simulink library "DAMA_lib"  (Simulink 6.6)
undefined symbols (not defined in the file or in its folder): aa2rot, D, DiscIntNeverNeededParam, DRprogressbar, epsilon, Kd, Ko, Kp, manip, manipulator, path_des, Q, q0, q_d0, rho, robot, show_3D, StartTime, subs, Ts, VR_handle, vrmfunc
libraries: DAMA_lib x7, vrlib x1, simulink x1
(part 3 of 4)

== system DAMA_lib/Kinematics/Transpose Jacobian Inverse Kinematics/Subsystem/Subsystem1 ==
  nsa_e_d_V : Inport
  Mux : Mux  Inputs=3
  invL1 : Fcn  Expr=2*(u(10)^2*u(1)^2+u(13)^2*u(4)^2+u(16)^2*u(7)^2+u(12)*u(3)*u(10)*u(1)+u(12)*u(3)*u(14)*u(5)+u(12)*u(3)*u(13)*u(4)+u(12)*u(3)*u(17)*u(8)+u(12)*u(3)*u(16)*u(7)+u(10)*u(1)*u(11)*u(2)+u(10)*u(1)*u(14)*u(5)+2*u(10)*u(1)*u(13)*u(4)+u(10)*u(1)*u(17)*u(8)+2*u(10)*u(1)*u(16)*u(7)+u(15)*u(6)*u(11)*u(2)+u(15)*u(6)*u(10)*u(1)+u(15)*u(6)*u(13)*u(4)+u(15)*u(6)*u(17)*u(8)+u(15)*u(6)*u(16)*u(7)+u(13)*u(4)*u(11)*u(2)+u(13)*u(4)*u(14)*u(5)+u(13)*u(4)*u(17)*u(8)+2*u(13)*u(4)*u(16)*u(7)+u(18)*u(9)*u(11)*u(2)+u(18)*u(9)*u(10)*u(1)+u(18)*u(9)*u(14)*u(5)+u(18)*u(9)*u(13)*u(4)+u(18)*u(9)*u(16)*u(7)+u(16)*u(7)*u(11)*u(2)+u(16)*u(7)*u(14)*u(5)+u(16)*u(7)*u(17)*u(8)-u(12)*u(2)*u(14)*u(6)-u(12)*u(2)*u(17)*u(9)-u(15)*u(5)*u(11)*u(3)-u(15)*u(5)*u(17)*u(9)-u(18)*u(8)*u(11)*u(3)-u(18)*u(8)*u(14)*u(6))/(u(12)*u(3)*u(13)^2*u(4)^2+u(12)*u(3)*u(16)^2*u(7)^2+u(12)^2*u(3)^2*u(14)*u(5)+u(12)^2*u(3)^2*u(13)*u(4)+u(12)^2*u(3)^2*u(17)*u(8)+u(12)^2*u(3)^2*u(16)*u(7)+u(11)*u(2)*u(13)^2*u(4)^2+u(11)*u(2)*u(16)^2*u(7)^2+u(11)^2*u(2)^2*u(15)*u(6)+u(11)^2*u(2)^2*u(13)*u(4)+u(11)^2*u(2)^2*u(18)*u(9)+u(11)^2*u(2)^2*u(16)*u(7)+u(15)*u(6)*u(10)^2*u(1)^2+u(15)*u(6)*u(16)^2*u(7)^2+u(15)^2*u(6)^2*u(11)*u(2)+u(15)^2*u(6)^2*u(10)*u(1)+u(15)^2*u(6)^2*u(17)*u(8)+u(15)^2*u(6)^2*u(16)*u(7)+u(14)*u(5)*u(10)^2*u(1)^2+u(14)*u(5)*u(16)^2*u(7)^2+u(14)^2*u(5)^2*u(12)*u(3)+u(14)^2*u(5)^2*u(10)*u(1)+u(14)^2*u(5)^2*u(18)*u(9)+u(14)^2*u(5)^2*u(16)*u(7)+u(18)*u(9)*u(10)^2*u(1)^2+u(18)*u(9)*u(13)^2*u(4)^2+u(18)^2*u(9)^2*u(11)*u(2)+u(18)^2*u(9)^2*u(10)*u(1)+u(18)^2*u(9)^2*u(14)*u(5)+u(18)^2*u(9)^2*u(13)*u(4)+u(17)*u(8)*u(10)^2*u(1)^2+u(17)*u(8)*u(13)^2*u(4)^2+u(17)^2*u(8)^2*u(12)*u(3)+u(17)^2*u(8)^2*u(10)*u(1)+u(17)^2*u(8)^2*u(15)*u(6)+u(17)^2*u(8)^2*u(13)*u(4)-u(10)*u(2)*u(14)^2*u(4)*u(5)-u(10)*u(2)*u(14)*u(4)^2*u(13)-u(10)*u(2)*u(17)*u(7)^2*u(16)-u(10)*u(2)*u(17)^2*u(7)*u(8)-u(10)*u(2)^2*u(14)*u(4)*u(11)+2*u(12)*u(3)*u(10)*u(1)*u(14)*u(5)+u(12)*u(3)*u(10)*u(1)*u(13)*u(4)+2*u(12)*u(3)*u(10)*u(1)*u(17)*u(8)+u(12)*u(3)*u(10)*u(1)*u(16)*u(7)+u(12)*u(3)*u(15)*u(6)*u(11)*u(2)+u(12)*u(3)*u(15)*u(6)*u(10)*u(1)+u(12)*u(3)*u(15)*u(6)*u(13)*u(4)+2*u(12)*u(3)*u(15)*u(6)*u(17)*u(8)+2*u(12)*u(3)*u(15)*u(6)*u(16)*u(7)+2*u(12)*u(3)*u(13)*u(4)*u(11)*u(2)+2*u(12)*u(3)*u(13)*u(4)*u(14)*u(5)+2*u(12)*u(3)*u(13)*u(4)*u(17)*u(8)+2*u(12)*u(3)*u(13)*u(4)*u(16)*u(7)+u(12)*u(3)*u(18)*u(9)*u(11)*u(2)+u(12)*u(3)*u(18)*u(9)*u(10)*u(1)+2*u(12)*u(3)*u(18)*u(9)*u(14)*u(5)+2*u(12)*u(3)*u(18)*u(9)*u(13)*u(4)+u(12)*u(3)*u(18)*u(9)*u(16)*u(7)+2*u(12)*u(3)*u(16)*u(7)*u(11)*u(2)+2*u(12)*u(3)*u(16)*u(7)*u(14)*u(5)+2*u(12)*u(3)*u(16)*u(7)*u(17)*u(8)-u(12)^2*u(3)*u(2)*u(14)*u(6)-u(12)^2*u(3)*u(2)*u(17)*u(9)-u(12)*u(3)^2*u(15)*u(5)*u(11)-u(12)*u(3)*u(15)*u(5)*u(17)*u(9)-u(12)*u(3)^2*u(18)*u(8)*u(11)-u(12)*u(3)*u(18)*u(8)*u(14)*u(6)+u(11)*u(2)*u(12)*u(3)*u(14)*u(5)+u(11)*u(2)*u(12)*u(3)*u(17)*u(8)+u(11)*u(2)*u(10)*u(1)*u(14)*u(5)+u(11)*u(2)*u(10)*u(1)*u(13)*u(4)+u(11)*u(2)*u(10)*u(1)*u(17)*u(8)+u(11)*u(2)*u(10)*u(1)*u(16)*u(7)+2*u(11)*u(2)*u(15)*u(6)*u(10)*u(1)+2*u(11)*u(2)*u(15)*u(6)*u(13)*u(4)+2*u(11)*u(2)*u(15)*u(6)*u(17)*u(8)+2*u(11)*u(2)*u(15)*u(6)*u(16)*u(7)+u(11)*u(2)*u(13)*u(4)*u(14)*u(5)+2*u(11)*u(2)*u(13)*u(4)*u(17)*u(8)+2*u(11)*u(2)*u(13)*u(4)*u(16)*u(7)+2*u(11)*u(2)*u(18)*u(9)*u(10)*u(1)+2*u(11)*u(2)*u(18)*u(9)*u(14)*u(5)+2*u(11)*u(2)*u(18)*u(9)*u(13)*u(4)+2*u(11)*u(2)*u(18)*u(9)*u(16)*u(7)+2*u(11)*u(2)*u(16)*u(7)*u(14)*u(5)+u(11)*u(2)*u(16)*u(7)*u(17)*u(8)-u(11)*u(2)^2*u(12)*u(14)*u(6)-u(11)*u(2)^2*u(12)*u(17)*u(9)-u(11)^2*u(2)*u(15)*u(5)*u(3)-u(11)*u(2)*u(15)*u(5)*u(17)*u(9)-u(11)^2*u(2)*u(18)*u(8)*u(3)-u(11)*u(2)*u(18)*u(8)*u(14)*u(6)+u(15)*u(6)*u(12)*u(3)*u(14)*u(5)+2*u(15)*u(6)*u(10)*u(1)*u(14)*u(5)+u(15)*u(6)*u(10)*u(1)*u(13)*u(4)+2*u(15)*u(6)*u(10)*u(1)*u(17)*u(8)+2*u(15)*u(6)*u(10)*u(1)*u(16)*u(7)+2*u(15)*u(6)*u(13)*u(4)*u(17)*u(8)+u(15)*u(6)*u(13)*u(4)*u(16)*u(7)+2*u(15)*u(6)*u(18)*u(9)*u(11)*u(2)+2*u(15)*u(6)*u(18)*u(9)*u(10)*u(1)+u(15)*u(6)*u(18)*u(9)*u(14)*u(5)+u(15)*u(6)*u(18)*u(9)*u(13)*u(4)+u(15)*u(6)*u(18)*u(9)*u(16)*u(7)+2*u(15)*u(6)*u(16)*u(7)*u(14)*u(5)+2*u(15)*u(6)*u(16)*u(7)*u(17)*u(8)-u(15)*u(6)^2*u(12)*u(2)*u(14)-u(15)*u(6)*u(12)*u(2)*u(17)*u(9)-u(15)^2*u(6)*u(5)*u(11)*u(3)-u(15)^2*u(6)*u(5)*u(17)*u(9)-u(15)*u(6)*u(18)*u(8)*u(11)*u(3)-u(15)*u(6)^2*u(18)*u(8)*u(14)+2*u(14)*u(5)*u(12)*u(3)*u(17)*u(8)+u(14)*u(5)*u(10)*u(1)*u(13)*u(4)+2*u(14)*u(5)*u(10)*u(1)*u(17)*u(8)+2*u(14)*u(5)*u(10)*u(1)*u(16)*u(7)+u(14)*u(5)*u(15)*u(6)*u(11)*u(2)+u(14)*u(5)*u(15)*u(6)*u(17)*u(8)+u(14)*u(5)*u(13)*u(4)*u(17)*u(8)+u(14)*u(5)*u(13)*u(4)*u(16)*u(7)+2*u(14)*u(5)*u(18)*u(9)*u(10)*u(1)+2*u(14)*u(5)*u(18)*u(9)*u(13)*u(4)+2*u(14)*u(5)*u(18)*u(9)*u(16)*u(7)+u(14)*u(5)*u(16)*u(7)*u(17)*u(8)-u(14)^2*u(5)*u(12)*u(2)*u(6)-u(14)*u(5)*u(12)*u(2)*u(17)*u(9)-u(14)*u(5)^2*u(15)*u(11)*u(3)-u(14)*u(5)^2*u(15)*u(17)*u(9)-u(14)*u(5)*u(18)*u(8)*u(11)*u(3)-u(14)^2*u(5)*u(18)*u(8)*u(6)+u(18)*u(9)*u(12)*u(3)*u(17)*u(8)+2*u(18)*u(9)*u(10)*u(1)*u(13)*u(4)+2*u(18)*u(9)*u(10)*u(1)*u(17)*u(8)+u(18)*u(9)*u(10)*u(1)*u(16)*u(7)+u(18)*u(9)*u(15)*u(6)*u(17)*u(8)+2*u(18)*u(9)*u(13)*u(4)*u(17)*u(8)+u(18)*u(9)*u(13)*u(4)*u(16)*u(7)-u(18)*u(9)*u(12)*u(2)*u(14)*u(6)-u(18)*u(9)^2*u(12)*u(2)*u(17)-u(18)*u(9)*u(15)*u(5)*u(11)*u(3)-u(18)*u(9)^2*u(15)*u(5)*u(17)-u(18)^2*u(9)*u(8)*u(11)*u(3)-u(18)^2*u(9)*u(8)*u(14)*u(6)+2*u(17)*u(8)*u(10)*u(1)*u(13)*u(4)+u(17)*u(8)*u(10)*u(1)*u(16)*u(7)+u(17)*u(8)*u(13)*u(4)*u(16)*u(7)+u(17)*u(8)*u(18)*u(9)*u(11)*u(2)+u(17)*u(8)*u(18)*u(9)*u(14)*u(5)-u(17)*u(8)*u(12)*u(2)*u(14)*u(6)-u(17)^2*u(8)*u(12)*u(2)*u(9)-u(17)*u(8)*u(15)*u(5)*u(11)*u(3)-u(17)^2*u(8)*u(15)*u(5)*u(9)-u(17)*u(8)^2*u(18)*u(11)*u(3)-u(17)*u(8)^2*u(18)*u(14)*u(6)-u(10)^2*u(2)*u(14)*u(4)*u(1)-u(10)*u(2)*u(14)*u(4)*u(17)*u(8)-u(10)*u(2)*u(14)*u(4)*u(16)*u(7)-u(10)*u(2)^2*u(17)*u(7)*u(11)-u(10)^2*u(2)*u(17)*u(7)*u(1)-u(10)*u(2)*u(17)*u(7)*u(14)*u(5)-u(10)*u(2)*u(17)*u(7)*u(13)*u(4)-u(10)*u(2)*u(12)*u(1)*u(14)*u(6)-u(10)*u(2)*u(12)*u(1)*u(17)*u(9)-u(10)*u(2)*u(15)*u(4)*u(11)*u(3)-u(10)*u(2)*u(15)*u(4)*u(14)*u(6)-u(10)*u(2)*u(15)*u(4)*u(17)*u(9)-u(10)*u(2)*u(18)*u(7)*u(11)*u(3)-u(10)*u(2)*u(18)*u(7)*u(14)*u(6)-u(10)*u(2)*u(18)*u(7)*u(17)*u(9)-u(13)*u(5)*u(11)^2*u(1)*u(2)-u(13)*u(5)*u(11)*u(1)^2*u(10)-u(13)*u(5)*u(17)*u(7)^2*u(16)-u(13)*u(5)*u(17)^2*u(7)*u(8)-u(13)*u(5)^2*u(11)*u(1)*u(14)-u(13)^2*u(5)*u(11)*u(1)*u(4)-u(13)*u(5)*u(11)*u(1)*u(17)*u(8)-u(13)*u(5)*u(11)*u(1)*u(16)*u(7)-u(13)*u(5)*u(17)*u(7)*u(11)*u(2)-u(13)*u(5)*u(17)*u(7)*u(10)*u(1)-u(13)*u(5)^2*u(17)*u(7)*u(14)-u(13)^2*u(5)*u(17)*u(7)*u(4)-u(13)*u(5)*u(12)*u(1)*u(11)*u(3)-u(13)*u(5)*u(12)*u(1)*u(14)*u(6)-u(13)*u(5)*u(12)*u(1)*u(17)*u(9)-u(13)*u(5)*u(15)*u(4)*u(11)*u(3)-u(13)*u(5)*u(15)*u(4)*u(17)*u(9)-u(13)*u(5)*u(18)*u(7)*u(11)*u(3)-u(13)*u(5)*u(18)*u(7)*u(14)*u(6)-u(13)*u(5)*u(18)*u(7)*u(17)*u(9)-u(16)*u(8)*u(14)^2*u(4)*u(5)-u(16)*u(8)*u(11)^2*u(1)*u(2)-u(16)*u(8)*u(14)*u(4)^2*u(13)-u(16)*u(8)*u(11)*u(1)^2*u(10)-u(16)*u(8)*u(11)*u(1)*u(14)*u(5)-u(16)*u(8)*u(11)*u(1)*u(13)*u(4)-u(16)*u(8)^2*u(11)*u(1)*u(17)-u(16)^2*u(8)*u(11)*u(1)*u(7)-u(16)*u(8)*u(14)*u(4)*u(11)*u(2)-u(16)*u(8)*u(14)*u(4)*u(10)*u(1)-u(16)*u(8)^2*u(14)*u(4)*u(17)-u(16)^2*u(8)*u(14)*u(4)*u(7)-u(16)*u(8)*u(12)*u(1)*u(11)*u(3)-u(16)*u(8)*u(12)*u(1)*u(14)*u(6)-u(16)*u(8)*u(12)*u(1)*u(17)*u(9)-u(16)*u(8)*u(15)*u(4)*u(11)*u(3)-u(16)*u(8)*u(15)*u(4)*u(14)*u(6)-u(16)*u(8)*u(15)*u(4)*u(17)*u(9)-u(16)*u(8)*u(18)*u(7)*u(11)*u(3)-u(16)*u(8)*u(18)*u(7)*u(14)*u(6)-u(10)*u(3)*u(15)^2*u(4)*u(6)-u(10)*u(3)*u(15)*u(4)^2*u(13)-u(10)*u(3)*u(18)^2*u(7)*u(9)-u(10)*u(3)*u(18)*u(7)^2*u(16)-u(10)*u(3)*u(11)*u(1)*u(15)*u(5)-u(10)*u(3)*u(11)*u(1)*u(18)*u(8)-u(10)*u(3)*u(14)*u(4)*u(12)*u(2)-u(10)*u(3)*u(14)*u(4)*u(15)*u(5)-u(10)*u(3)*u(14)*u(4)*u(18)*u(8)-u(10)*u(3)*u(17)*u(7)*u(12)*u(2)-u(10)*u(3)*u(17)*u(7)*u(15)*u(5)-u(10)*u(3)*u(17)*u(7)*u(18)*u(8)-u(10)*u(3)^2*u(15)*u(4)*u(12)-u(10)^2*u(3)*u(15)*u(4)*u(1)-u(10)*u(3)*u(15)*u(4)*u(18)*u(9)-u(10)*u(3)*u(15)*u(4)*u(16)*u(7)-u(10)*u(3)^2*u(18)*u(7)*u(12)-u(10)^2*u(3)*u(18)*u(7)*u(1)-u(10)*u(3)*u(18)*u(7)*u(15)*u(6)-u(10)*u(3)*u(18)*u(7)*u(13)*u(4)-u(13)*u(6)*u(12)*u(1)^2*u(10)-u(13)*u(6)*u(12)^2*u(1)*u(3)-u(13)*u(6)*u(18)^2*u(7)*u(9)-u(13)*u(6)*u(18)*u(7)^2*u(16)-u(13)*u(6)*u(11)*u(1)*u(12)*u(2)-u(13)*u(6)*u(11)*u(1)*u(15)*u(5)-u(13)*u(6)*u(11)*u(1)*u(18)*u(8)-u(13)*u(6)*u(14)*u(4)*u(12)*u(2)-u(13)*u(6)*u(14)*u(4)*u(18)*u(8)-u(13)*u(6)*u(17)*u(7)*u(12)*u(2)-u(13)*u(6)*u(17)*u(7)*u(15)*u(5)-u(13)*u(6)*u(17)*u(7)*u(18)*u(8)-u(13)*u(6)^2*u(12)*u(1)*u(15)-u(13)^2*u(6)*u(12)*u(1)*u(4)-u(13)*u(6)*u(12)*u(1)*u(18)*u(9)-u(13)*u(6)*u(12)*u(1)*u(16)*u(7)-u(13)*u(6)*u(18)*u(7)*u(12)*u(3)-u(13)*u(6)*u(18)*u(7)*u(10)*u(1)-u(13)*u(6)^2*u(18)*u(7)*u(15)-u(13)^2*u(6)*u(18)*u(7)*u(4)-u(16)*u(9)*u(12)*u(1)^2*u(10)-u(16)*u(9)*u(12)^2*u(1)*u(3)-u(16)*u(9)*u(15)^2*u(4)*u(6)-u(16)*u(9)*u(15)*u(4)^2*u(13)-u(16)*u(9)*u(11)*u(1)*u(12)*u(2)-u(16)*u(9)*u(11)*u(1)*u(15)*u(5)-u(16)*u(9)*u(11)*u(1)*u(18)*u(8)-u(16)*u(9)*u(14)*u(4)*u(12)*u(2)-u(16)*u(9)*u(14)*u(4)*u(15)*u(5)-u(16)*u(9)*u(14)*u(4)*u(18)*u(8)-u(16)*u(9)*u(17)*u(7)*u(12)*u(2)-u(16)*u(9)*u(17)*u(7)*u(15)*u(5)-u(16)*u(9)*u(12)*u(1)*u(15)*u(6)-u(16)*u(9)*u(12)*u(1)*u(13)*u(4)-u(16)*u(9)^2*u(12)*u(1)*u(18)-u(16)^2*u(9)*u(12)*u(1)*u(7)-u(16)*u(9)*u(15)*u(4)*u(12)*u(3)-u(16)*u(9)*u(15)*u(4)*u(10)*u(1)-u(16)*u(9)^2*u(15)*u(4)*u(18)-u(16)^2*u(9)*u(15)*u(4)*u(7))*u(19)+2*(u(14)^2*u(4)*u(5)+u(11)^2*u(1)*u(2)+u(14)*u(4)^2*u(13)+u(11)*u(1)^2*u(10)+u(17)*u(7)^2*u(16)+u(17)^2*u(7)*u(8)+u(11)*u(1)*u(14)*u(5)+u(11)*u(1)*u(13)*u(4)+u(11)*u(1)*u(17)*u(8)+u(11)*u(1)*u(16)*u(7)+u(14)*u(4)*u(11)*u(2)+u(14)*u(4)*u(10)*u(1)+u(14)*u(4)*u(17)*u(8)+u(14)*u(4)*u(16)*u(7)+u(17)*u(7)*u(11)*u(2)+u(17)*u(7)*u(10)*u(1)+u(17)*u(7)*u(14)*u(5)+u(17)*u(7)*u(13)*u(4)+u(12)*u(1)*u(11)*u(3)+u(12)*u(1)*u(14)*u(6)+u(12)*u(1)*u(17)*u(9)+u(15)*u(4)*u(11)*u(3)+u(15)*u(4)*u(14)*u(6)+u(15)*u(4)*u(17)*u(9)+u(18)*u(7)*u(11)*u(3)+u(18)*u(7)*u(14)*u(6)+u(18)*u(7)*u(17)*u(9))/(u(12)*u(3)*u(13)^2*u(4)^2+u(12)*u(3)*u(16)^2*u(7)^2+u(12)^2*u(3)^2*u(14)*u(5)+u(12)^2*u(3)^2*u(13)*u(4)+u(12)^2*u(3)^2*u(17)*u(8)+u(12)^2*u(3)^2*u(16)*u(7)+u(11)*u(2)*u(13)^2*u(4)^2+u(11)*u(2)*u(16)^2*u(7)^2+u(11)^2*u(2)^2*u(15)*u(6)+u(11)^2*u(2)^2*u(13)*u(4)+u(11)^2*u(2)^2*u(18)*u(9)+u(11)^2*u(2)^2*u(16)*u(7)+u(15)*u(6)*u(10)^2*u(1)^2+u(15)*u(6)*u(16)^2*u(7)^2+u(15)^2*u(6)^2*u(11)*u(2)+u(15)^2*u(6)^2*u(10)*u(1)+u(15)^2*u(6)^2*u(17)*u(8)+u(15)^2*u(6)^2*u(16)*u(7)+u(14)*u(5)*u(10)^2*u(1)^2+u(14)*u(5)*u(16)^2*u(7)^2+u(14)^2*u(5)^2*u(12)*u(3)+u(14)^2*u(5)^2*u(10)*u(1)+u(14)^2*u(5)^2*u(18)*u(9)+u(14)^2*u(5)^2*u(16)*u(7)+u(18)*u(9)*u(10)^2*u(1)^2+u(18)*u(9)*u(13)^2*u(4)^2+u(18)^2*u(9)^2*u(11)*u(2)+u(18)^2*u(9)^2*u(10)*u(1)+u(18)^2*u(9)^2*u(14)*u(5)+u(18)^2*u(9)^2*u(13)*u(4)+u(17)*u(8)*u(10)^2*u(1)^2+u(17)*u(8)*u(13)^2*u(4)^2+u(17)^2*u(8)^2*u(12)*u(3)+u(17)^2*u(8)^2*u(10)*u(1)+u(17)^2*u(8)^2*u(15)*u(6)+u(17)^2*u(8)^2*u(13)*u(4)-u(10)*u(2)*u(14)^2*u(4)*u(5)-u(10)*u(2)*u(14)*u(4)^2*u(13)-u(10)*u(2)*u(17)*u(7)^2*u(16)-u(10)*u(2)*u(17)^2*u(7)*u(8)-u(10)*u(2)^2*u(14)*u(4)*u(11)+2*u(12)*u(3)*u(10)*u(1)*u(14)*u(5)+u(12)*u(3)*u(10)*u(1)*u(13)*u(4)+2*u(12)*u(3)*u(10)*u(1)*u(17)*u(8)+u(12)*u(3)*u(10)*u(1)*u(16)*u(7)+u(12)*u(3)*u(15)*u(6)*u(11)*u(2)+u(12)*u(3)*u(15)*u(6)*u(10)*u(1)+u(12)*u(3)*u(15)*u(6)*u(13)*u(4)+2*u(12)*u(3)*u(15)*u(6)*u(17)*u(8)+2*u(12)*u(3)*u(15)*u(6)*u(16)*u(7)+2*u(12)*u(3)*u(13)*u(4)*u(11)*u(2)+2*u(12)*u(3)*u(13)*u(4)*u(14)*u(5)+2*u(12)*u(3)*u(13)*u(4)*u(17)*u(8)+2*u(12)*u(3)*u(13)*u(4)*u(16)*u(7)+u(12)*u(3)*u(18)*u(9)*u(11)*u(2)+u(12)*u(3)*u(18)*u(9)*u(10)*u(1)+2*u(12)*u(3)*u(18)*u(9)*u(14)*u(5)+2*u(12)*u(3)*u(18)*u(9)*u(13)*u(4)+u(12)*u(3)*u(18)*u(9)*u(16)*u(7)+2*u(12)*u(3)*u(16)*u(7)*u(11)*u(2)+2*u(12)*u(3)*u(16)*u(7)*u(14)*u(5)+2*u(12)*u(3)*u(16)*u(7)*u(17)*u(8)-u(12)^2*u(3)*u(2)*u(14)*u(6)-u(12)^2*u(3)*u(2)*u(17)*u(9)-u(12)*u(3)^2*u(15)*u(5)*u(11)-u(12)*u(3)*u(15)*u(5)*u(17)*u(9)-u(12)*u(3)^2*u(18)*u(8)*u(11)-u(12)*u(3)*u(18)*u(8)*u(14)*u(6)+u(11)*u(2)*u(12)*u(3)*u(14)*u(5)+u(11)*u(2)*u(12)*u(3)*u(17)*u(8)+u(11)*u(2)*u(10)*u(1)*u(14)*u(5)+u(11)*u(2)*u(10)*u(1)*u(13)*u(4)+u(11)*u(2)*u(10)*u(1)*u(17)*u(8)+u(11)*u(2)*u(10)*u(1)*u(16)*u(7)+2*u(11)*u(2)*u(15)*u(6)*u(10)*u(1)+2*u(11)*u(2)*u(15)*u(6)*u(13)*u(4)+2*u(11)*u(2)*u(15)*u(6)*u(17)*u(8)+2*u(11)*u(2)*u(15)*u(6)*u(16)*u(7)+u(11)*u(2)*u(13)*u(4)*u(14)*u(5)+2*u(11)*u(2)*u(13)*u(4)*u(17)*u(8)+2*u(11)*u(2)*u(13)*u(4)*u(16)*u(7)+2*u(11)*u(2)*u(18)*u(9)*u(10)*u(1)+2*u(11)*u(2)*u(18)*u(9)*u(14)*u(5)+2*u(11)*u(2)*u(18)*u(9)*u(13)*u(4)+2*u(11)*u(2)*u(18)*u(9)*u(16)*u(7)+2*u(11)*u(2)*u(16)*u(7)*u(14)*u(5)+u(11)*u(2)*u(16)*u(7)*u(17)*u(8)-u(11)*u(2)^2*u(12)*u(14)*u(6)-u(11)*u(2)^2*u(12)*u(17)*u(9)-u(11)^2*u(2)*u(15)*u(5)*u(3)-u(11)*u(2)*u(15)*u(5)*u(17)*u(9)-u(11)^2*u(2)*u(18)*u(8)*u(3)-u(11)*u(2)*u(18)*u(8)*u(14)*u(6)+u(15)*u(6)*u(12)*u(3)*u(14)*u(5)+2*u(15)*u(6)*u(10)*u(1)*u(14)*u(5)+u(15)*u(6)*u(10)*u(1)*u(13)*u(4)+2*u(15)*u(6)*u(10)*u(1)*u(17)*u(8)+2*u(15)*u(6)*u(10)*u(1)*u(16)*u(7)+2*u(15)*u(6)*u(13)*u(4)*u(17)*u(8)+u(15)*u(6)*u(13)*u(4)*u(16)*u(7)+2*u(15)*u(6)*u(18)*u(9)*u(11)*u(2)+2*u(15)*u(6)*u(18)*u(9)*u(10)*u(1)+u(15)*u(6)*u(18)*u(9)*u(14)*u(5)+u(15)*u(6)*u(18)*u(9)*u(13)*u(4)+u(15)*u(6)*u(18)*u(9)*u(16)*u(7)+2*u(15)*u(6)*u(16)*u(7)*u(14)*u(5)+2*u(15)*u(6)*u(16)*u(7)*u(17)*u(8)-u(15)*u(6)^2*u(12)*u(2)*u(14)-u(15)*u(6)*u(12)*u(2)*u(17)*u(9)-u(15)^2*u(6)*u(5)*u(11)*u(3)-u(15)^2*u(6)*u(5)*u(17)*u(9)-u(15)*u(6)*u(18)*u(8)*u(11)*u(3)-u(15)*u(6)^2*u(18)*u(8)*u(14)+2*u(14)*u(5)*u(12)*u(3)*u(17)*u(8)+u(14)*u(5)*u(10)*u(1)*u(13)*u(4)+2*u(14)*u(5)*u(10)*u(1)*u(17)*u(8)+2*u(14)*u(5)*u(10)*u(1)*u(16)*u(7)+u(14)*u(5)*u(15)*u(6)*u(11)*u(2)+u(14)*u(5)*u(15)*u(6)*u(17)*u(8)+u(14)*u(5)*u(13)*u(4)*u(17)*u(8)+u(14)*u(5)*u(13)*u(4)*u(16)*u(7)+2*u(14)*u(5)*u(18)*u(9)*u(10)*u(1)+2*u(14)*u(5)*u(18)*u(9)*u(13)*u(4)+2*u(14)*u(5)*u(18)*u(9)*u(16)*u(7)+u(14)*u(5)*u(16)*u(7)*u(17)*u(8)-u(14)^2*u(5)*u(12)*u(2)*u(6)-u(14)*u(5)*u(12)*u(2)*u(17)*u(9)-u(14)*u(5)^2*u(15)*u(11)*u(3)-u(14)*u(5)^2*u(15)*u(17)*u(9)-u(14)*u(5)*u(18)*u(8)*u(11)*u(3)-u(14)^2*u(5)*u(18)*u(8)*u(6)+u(18)*u(9)*u(12)*u(3)*u(17)*u(8)+2*u(18)*u(9)*u(10)*u(1)*u(13)*u(4)+2*u(18)*u(9)*u(10)*u(1)*u(17)*u(8)+u(18)*u(9)*u(10)*u(1)*u(16)*u(7)+u(18)*u(9)*u(15)*u(6)*u(17)*u(8)+2*u(18)*u(9)*u(13)*u(4)*u(17)*u(8)+u(18)*u(9)*u(13)*u(4)*u(16)*u(7)-u(18)*u(9)*u(12)*u(2)*u(14)*u(6)-u(18)*u(9)^2*u(12)*u(2)*u(17)-u(18)*u(9)*u(15)*u(5)*u(11)*u(3)-u(18)*u(9)^2*u(15)*u(5)*u(17)-u(18)^2*u(9)*u(8)*u(11)*u(3)-u(18)^2*u(9)*u(8)*u(14)*u(6)+2*u(17)*u(8)*u(10)*u(1)*u(13)*u(4)+u(17)*u(8)*u(10)*u(1)*u(16)*u(7)+u(17)*u(8)*u(13)*u(4)*u(16)*u(7)+u(17)*u(8)*u(18)*u(9)*u(11)*u(2)+u(17)*u(8)*u(18)*u(9)*u(14)*u(5)-u(17)*u(8)*u(12)*u(2)*u(14)*u(6)-u(17)^2*u(8)*u(12)*u(2)*u(9)-u(17)*u(8)*u(15)*u(5)*u(11)*u(3)-u(17)^2*u(8)*u(15)*u(5)*u(9)-u(17)*u(8)^2*u(18)*u(11)*u(3)-u(17)*u(8)^2*u(18)*u(14)*u(6)-u(10)^2*u(2)*u(14)*u(4)*u(1)-u(10)*u(2)*u(14)*u(4)*u(17)*u(8)-u(10)*u(2)*u(14)*u(4)*u(16)*u(7)-u(10)*u(2)^2*u(17)*u(7)*u(11)-u(10)^2*u(2)*u(17)*u(7)*u(1)-u(10)*u(2)*u(17)*u(7)*u(14)*u(5)-u(10)*u(2)*u(17)*u(7)*u(13)*u(4)-u(10)*u(2)*u(12)*u(1)*u(14)*u(6)-u(10)*u(2)*u(12)*u(1)*u(17)*u(9)-u(10)*u(2)*u(15)*u(4)*u(11)*u(3)-u(10)*u(2)*u(15)*u(4)*u(14)*u(6)-u(10)*u(2)*u(15)*u(4)*u(17)*u(9)-u(10)*u(2)*u(18)*u(7)*u(11)*u(3)-u(10)*u(2)*u(18)*u(7)*u(14)*u(6)-u(10)*u(2)*u(18)*u(7)*u(17)*u(9)-u(13)*u(5)*u(11)^2*u(1)*u(2)-u(13)*u(5)*u(11)*u(1)^2*u(10)-u(13)*u(5)*u(17)*u(7)^2*u(16)-u(13)*u(5)*u(17)^2*u(7)*u(8)-u(13)*u(5)^2*u(11)*u(1)*u(14)-u(13)^2*u(5)*u(11)*u(1)*u(4)-u(13)*u(5)*u(11)*u(1)*u(17)*u(8)-u(13)*u(5)*u(11)*u(1)*u(16)*u(7)-u(13)*u(5)*u(17)*u(7)*u(11)*u(2)-u(13)*u(5)*u(17)*u(7)*u(10)*u(1)-u(13)*u(5)^2*u(17)*u(7)*u(14)-u(13)^2*u(5)*u(17)*u(7)*u(4)-u(13)*u(5)*u(12)*u(1)*u(11)*u(3)-u(13)*u(5)*u(12)*u(1)*u(14)*u(6)-u(13)*u(5)*u(12)*u(1)*u(17)*u(9)-u(13)*u(5)*u(15)*u(4)*u(11)*u(3)-u(13)*u(5)*u(15)*u(4)*u(17)*u(9)-u(13)*u(5)*u(18)*u(7)*u(11)*u(3)-u(13)*u(5)*u(18)*u(7)*u(14)*u(6)-u(13)*u(5)*u(18)*u(7)*u(17)*u(9)-u(16)*u(8)*u(14)^2*u(4)*u(5)-u(16)*u(8)*u(11)^2*u(1)*u(2)-u(16)*u(8)*u(14)*u(4)^2*u(13)-u(16)*u(8)*u(11)*u(1)^2*u(10)-u(16)*u(8)*u(11)*u(1)*u(14)*u(5)-u(16)*u(8)*u(11)*u(1)*u(13)*u(4)-u(16)*u(8)^2*u(11)*u(1)*u(17)-u(16)^2*u(8)*u(11)*u(1)*u(7)-u(16)*u(8)*u(14)*u(4)*u(11)*u(2)-u(16)*u(8)*u(14)*u(4)*u(10)*u(1)-u(16)*u(8)^2*u(14)*u(4)*u(17)-u(16)^2*u(8)*u(14)*u(4)*u(7)-u(16)*u(8)*u(12)*u(1)*u(11)*u(3)-u(16)*u(8)*u(12)*u(1)*u(14)*u(6)-u(16)*u(8)*u(12)*u(1)*u(17)*u(9)-u(16)*u(8)*u(15)*u(4)*u(11)*u(3)-u(16)*u(8)*u(15)*u(4)*u(14)*u(6)-u(16)*u(8)*u(15)*u(4)*u(17)*u(9)-u(16)*u(8)*u(18)*u(7)*u(11)*u(3)-u(16)*u(8)*u(18)*u(7)*u(14)*u(6)-u(10)*u(3)*u(15)^2*u(4)*u(6)-u(10)*u(3)*u(15)*u(4)^2*u(13)-u(10)*u(3)*u(18)^2*u(7)*u(9)-u(10)*u(3)*u(18)*u(7)^2*u(16)-u(10)*u(3)*u(11)*u(1)*u(15)*u(5)-u(10)*u(3)*u(11)*u(1)*u(18)*u(8)-u(10)*u(3)*u(14)*u(4)*u(12)*u(2)-u(10)*u(3)*u(14)*u(4)*u(15)*u(5)-u(10)*u(3)*u(14)*u(4)*u(18)*u(8)-u(10)*u(3)*u(17)*u(7)*u(12)*u(2)-u(10)*u(3)*u(17)*u(7)*u(15)*u(5)-u(10)*u(3)*u(17)*u(7)*u(18)*u(8)-u(10)*u(3)^2*u(15)*u(4)*u(12)-u(10)^2*u(3)*u(15)*u(4)*u(1)-u(10)*u(3)*u(15)*u(4)*u(18)*u(9)-u(10)*u(3)*u(15)*u(4)*u(16)*u(7)-u(10)*u(3)^2*u(18)*u(7)*u(12)-u(10)^2*u(3)*u(18)*u(7)*u(1)-u(10)*u(3)*u(18)*u(7)*u(15)*u(6)-u(10)*u(3)*u(18)*u(7)*u(13)*u(4)-u(13)*u(6)*u(12)*u(1)^2*u(10)-u(13)*u(6)*u(12)^2*u(1)*u(3)-u(13)*u(6)*u(18)^2*u(7)*u(9)-u(13)*u(6)*u(18)*u(7)^2*u(16)-u(13)*u(6)*u(11)*u(1)*u(12)*u(2)-u(13)*u(6)*u(11)*u(1)*u(15)*u(5)-u(13)*u(6)*u(11)*u(1)*u(18)*u(8)-u(13)*u(6)*u(14)*u(4)*u(12)*u(2)-u(13)*u(6)*u(14)*u(4)*u(18)*u(8)-u(13)*u(6)*u(17)*u(7)*u(12)*u(2)-u(13)*u(6)*u(17)*u(7)*u(15)*u(5)-u(13)*u(6)*u(17)*u(7)*u(18)*u(8)-u(13)*u(6)^2*u(12)*u(1)*u(15)-u(13)^2*u(6)*u(12)*u(1)*u(4)-u(13)*u(6)*u(12)*u(1)*u(18)*u(9)-u(13)*u(6)*u(12)*u(1)*u(16)*u(7)-u(13)*u(6)*u(18)*u(7)*u(12)*u(3)-u(13)*u(6)*u(18)*u(7)*u(10)*u(1)-u(13)*u(6)^2*u(18)*u(7)*u(15)-u(13)^2*u(6)*u(18)*u(7)*u(4)-u(16)*u(9)*u(12)*u(1)^2*u(10)-u(16)*u(9)*u(12)^2*u(1)*u(3)-u(16)*u(9)*u(15)^2*u(4)*u(6)-u(16)*u(9)*u(15)*u(4)^2*u(13)-u(16)*u(9)*u(11)*u(1)*u(12)*u(2)-u(16)*u(9)*u(11)*u(1)*u(15)*u(5)-u(16)*u(9)*u(11)*u(1)*u(18)*u(8)-u(16)*u(9)*u(14)*u(4)*u(12)*u(2)-u(16)*u(9)*u(14)*u(4)*u(15)*u(5)-u(16)*u(9)*u(14)*u(4)*u(18)*u(8)-u(16)*u(9)*u(17)*u(7)*u(12)*u(2)-u(16)*u(9)*u(17)*u(7)*u(15)*u(5)-u(16)*u(9)*u(12)*u(1)*u(15)*u(6)-u(16)*u(9)*u(12)*u(1)*u(13)*u(4)-u(16)*u(9)^2*u(12)*u(1)*u(18)-u(16)^2*u(9)*u(12)*u(1)*u(7)-u(16)*u(9)*u(15)*u(4)*u(12)*u(3)-u(16)*u(9)*u(15)*u(4)*u(10)*u(1)-u(16)*u(9)^2*u(15)*u(4)*u(18)-u(16)^2*u(9)*u(15)*u(4)*u(7))*u(20)+2*(u(12)*u(1)^2*u(10)+u(12)^2*u(1)*u(3)+u(15)^2*u(4)*u(6)+u(15)*u(4)^2*u(13)+u(18)^2*u(7)*u(9)+u(18)*u(7)^2*u(16)+u(11)*u(1)*u(12)*u(2)+u(11)*u(1)*u(15)*u(5)+u(11)*u(1)*u(18)*u(8)+u(14)*u(4)*u(12)*u(2)+u(14)*u(4)*u(15)*u(5)+u(14)*u(4)*u(18)*u(8)+u(17)*u(7)*u(12)*u(2)+u(17)*u(7)*u(15)*u(5)+u(17)*u(7)*u(18)*u(8)+u(12)*u(1)*u(15)*u(6)+u(12)*u(1)*u(13)*u(4)+u(12)*u(1)*u(18)*u(9)+u(12)*u(1)*u(16)*u(7)+u(15)*u(4)*u(12)*u(3)+u(15)*u(4)*u(10)*u(1)+u(15)*u(4)*u(18)*u(9)+u(15)*u(4)*u(16)*u(7)+u(18)*u(7)*u(12)*u(3)+u(18)*u(7)*u(10)*u(1)+u(18)*u(7)*u(15)*u(6)+u(18)*u(7)*u(13)*u(4))/(u(12)*u(3)*u(13)^2*u(4)^2+u(12)*u(3)*u(16)^2*u(7)^2+u(12)^2*u(3)^2*u(14)*u(5)+u(12)^2*u(3)^2*u(13)*u(4)+u(12)^2*u(3)^2*u(17)*u(8)+u(12)^2*u(3)^2*u(16)*u(7)+u(11)*u(2)*u(13)^2*u(4)^2+u(11)*u(2)*u(16)^2*u(7)^2+u(11)^2*u(2)^2*u(15)*u(6)+u(11)^2*u(2)^2*u(13)*u(4)+u(11)^2*u(2)^2*u(18)*u(9)+u(11)^2*u(2)^2*u(16)*u(7)+u(15)*u(6)*u(10)^2*u(1)^2+u(15)*u(6)*u(16)^2*u(7)^2+u(15)^2*u(6)^2*u(11)*u(2)+u(15)^2*u(6)^2*u(10)*u(1)+u(15)^2*u(6)^2*u(17)*u(8)+u(15)^2*u(6)^2*u(16)*u(7)+u(14)*u(5)*u(10)^2*u(1)^2+u(14)*u(5)*u(16)^2*u(7)^2+u(14)^2*u(5)^2*u(12)*u(3)+u(14)^2*u(5)^2*u(10)*u(1)+u(14)^2*u(5)^2*u(18)*u(9)+u(14)^2*u(5)^2*u(16)*u(7)+u(18)*u(9)*u(10)^2*u(1)^2+u(18)*u(9)*u(13)^2*u(4)^2+u(18)^2*u(9)^2*u(11)*u(2)+u(18)^2*u(9)^2*u(10)*u(1)+u(18)^2*u(9)^2*u(14)*u(5)+u(18)^2*u(9)^2*u(13)*u(4)+u(17)*u(8)*u(10)^2*u(1)^2+u(17)*u(8)*u(13)^2*u(4)^2+u(17)^2*u(8)^2*u(12)*u(3)+u(17)^2*u(8)^2*u(10)*u(1)+u(17)^2*u(8)^2*u(15)*u(6)+u(17)^2*u(8)^2*u(13)*u(4)-u(10)*u(2)*u(14)^2*u(4)*u(5)-u(10)*u(2)*u(14)*u(4)^2*u(13)-u(10)*u(2)*u(17)*u(7)^2*u(16)-u(10)*u(2)*u(17)^2*u(7)*u(8)-u(10)*u(2)^2*u(14)*u(4)*u(11)+2*u(12)*u(3)*u(10)*u(1)*u(14)*u(5)+u(12)*u(3)*u(10)*u(1)*u(13)*u(4)+2*u(12)*u(3)*u(10)*u(1)*u(17)*u(8)+u(12)*u(3)*u(10)*u(1)*u(16)*u(7)+u(12)*u(3)*u(15)*u(6)*u(11)*u(2)+u(12)*u(3)*u(15)*u(6)*u(10)*u(1)+u(12)*u(3)*u(15)*u(6)*u(13)*u(4)+2*u(12)*u(3)*u(15)*u(6)*u(17)*u(8)+2*u(12)*u(3)*u(15)*u(6)*u(16)*u(7)+2*u(12)*u(3)*u(13)*u(4)*u(11)*u(2)+2*u(12)*u(3)*u(13)*u(4)*u(14)*u(5)+2*u(12)*u(3)*u(13)*u(4)*u(17)*u(8)+2*u(12)*u(3)*u(13)*u(4)*u(16)*u(7)+u(12)*u(3)*u(18)*u(9)*u(11)*u(2)+u(12)*u(3)*u(18)*u(9)*u(10)*u(1)+2*u(12)*u(3)*u(18)*u(9)*u(14)*u(5)+2*u(12)*u(3)*u(18)*u(9)*u(13)*u(4)+u(12)*u(3)*u(18)*u(9)*u(16)*u(7)+2*u(12)*u(3)*u(16)*u(7)*u(11)*u(2)+2*u(12)*u(3)*u(16)*u(7)*u(14)*u(5)+2*u(12)*u(3)*u(16)*u(7)*u(17)*u(8)-u(12)^2*u(3)*u(2)*u(14)*u(6)-u(12)^2*u(3)*u(2)*u(17)*u(9)-u(12)*u(3)^2*u(15)*u(5)*u(11)-u(12)*u(3)*u(15)*u(5)*u(17)*u(9)-u(12)*u(3)^2*u(18)*u(8)*u(11)-u(12)*u(3)*u(18)*u(8)*u(14)*u(6)+u(11)*u(2)*u(12)*u(3)*u(14)*u(5)+u(11)*u(2)*u(12)*u(3)*u(17)*u(8)+u(11)*u(2)*u(10)*u(1)*u(14)*u(5)+u(11)*u(2)*u(10)*u(1)*u(13)*u(4)+u(11)*u(2)*u(10)*u(1)*u(17)*u(8)+u(11)*u(2)*u(10)*u(1)*u(16)*u(7)+2*u(11)*u(2)*u(15)*u(6)*u(10)*u(1)+2*u(11)*u(2)*u(15)*u(6)*u(13)*u(4)+2*u(11)*u(2)*u(15)*u(6)*u(17)*u(8)+2*u(11)*u(2)*u(15)*u(6)*u(16)*u(7)+u(11)*u(2)*u(13)*u(4)*u(14)*u(5)+2*u(11)*u(2)*u(13)*u(4)*u(17)*u(8)+2*u(11)*u(2)*u(13)*u(4)*u(16)*u(7)+2*u(11)*u(2)*u(18)*u(9)*u(10)*u(1)+2*u(11)*u(2)*u(18)*u(9)*u(14)*u(5)+2*u(11)*u(2)*u(18)*u(9)*u(13)*u(4)+2*u(11)*u(2)*u(18)*u(9)*u(16)*u(7)+2*u(11)*u(2)*u(16)*u(7)*u(14)*u(5)+u(11)*u(2)*u(16)*u(7)*u(17)*u(8)-u(11)*u(2)^2*u(12)*u(14)*u(6)-u(11)*u(2)^2*u(12)*u(17)*u(9)-u(11)^2*u(2)*u(15)*u(5)*u(3)-u(11)*u(2)*u(15)*u(5)*u(17)*u(9)-u(11)^2*u(2)*u(18)*u(8)*u(3)-u(11)*u(2)*u(18)*u(8)*u(14)*u(6)+u(15)*u(6)*u(12)*u(3)*u(14)*u(5)+2*u(15)*u(6)*u(10)*u(1)*u(14)*u(5)+u(15)*u(6)*u(10)*u(1)*u(13)*u(4)+2*u(15)*u(6)*u(10)*u(1)*u(17)*u(8)+2*u(15)*u(6)*u(10)*u(1)*u(16)*u(7)+2*u(15)*u(6)*u(13)*u(4)*u(17)*u(8)+u(15)*u(6)*u(13)*u(4)*u(16)*u(7)+2*u(15)*u(6)*u(18)*u(9)*u(11)*u(2)+2*u(15)*u(6)*u(18)*u(9)*u(10)*u(1)+u(15)*u(6)*u(18)*u(9)*u(14)*u(5)+u(15)*u(6)*u(18)*u(9)*u(13)*u(4)+u(15)*u(6)*u(18)*u(9)*u(16)*u(7)+2*u(15)*u(6)*u(16)*u(7)*u(14)*u(5)+2*u(15)*u(6)*u(16)*u(7)*u(17)*u(8)-u(15)*u(6)^2*u(12)*u(2)*u(14)-u(15)*u(6)*u(12)*u(2)*u(17)*u(9)-u(15)^2*u(6)*u(5)*u(11)*u(3)-u(15)^2*u(6)*u(5)*u(17)*u(9)-u(15)*u(6)*u(18)*u(8)*u(11)*u(3)-u(15)*u(6)^2*u(18)*u(8)*u(14)+2*u(14)*u(5)*u(12)*u(3)*u(17)*u(8)+u(14)*u(5)*u(10)*u(1)*u(13)*u(4)+2*u(14)*u(5)*u(10)*u(1)*u(17)*u(8)+2*u(14)*u(5)*u(10)*u(1)*u(16)*u(7)+u(14)*u(5)*u(15)*u(6)*u(11)*u(2)+u(14)*u(5)*u(15)*u(6)*u(17)*u(8)+u(14)*u(5)*u(13)*u(4)*u(17)*u(8)+u(14)*u(5)*u(13)*u(4)*u(16)*u(7)+2*u(14)*u(5)*u(18)*u(9)*u(10)*u(1)+2*u(14)*u(5)*u(18)*u(9)*u(13)*u(4)+2*u(14)*u(5)*u(18)*u(9)*u(16)*u(7)+u(14)*u(5)*u(16)*u(7)*u(17)*u(8)-u(14)^2*u(5)*u(12)*u(2)*u(6)-u(14)*u(5)*u(12)*u(2)*u(17)*u(9)-u(14)*u(5)^2*u(15)*u(11)*u(3)-u(14)*u(5)^2*u(15)*u(17)*u(9)-u(14)*u(5)*u(18)*u(8)*u(11)*u(3)-u(14)^2*u(5)*u(18)*u(8)*u(6)+u(18)*u(9)*u(12)*u(3)*u(17)*u(8)+2*u(18)*u(9)*u(10)*u(1)*u(13)*u(4)+2*u(18)*u(9)*u(10)*u(1)*u(17)*u(8)+u(18)*u(9)*u(10)*u(1)*u(16)*u(7)+u(18)*u(9)*u(15)*u(6)*u(17)*u(8)+2*u(18)*u(9)*u(13)*u(4)*u(17)*u(8)+u(18)*u(9)*u(13)*u(4)*u(16)*u(7)-u(18)*u(9)*u(12)*u(2)*u(14)*u(6)-u(18)*u(9)^2*u(12)*u(2)*u(17)-u(18)*u(9)*u(15)*u(5)*u(11)*u(3)-u(18)*u(9)^2*u(15)*u(5)*u(17)-u(18)^2*u(9)*u(8)*u(11)*u(3)-u(18)^2*u(9)*u(8)*u(14)*u(6)+2*u(17)*u(8)*u(10)*u(1)*u(13)*u(4)+u(17)*u(8)*u(10)*u(1)*u(16)*u(7)+u(17)*u(8)*u(13)*u(4)*u(16)*u(7)+u(17)*u(8)*u(18)*u(9)*u(11)*u(2)+u(17)*u(8)*u(18)*u(9)*u(14)*u(5)-u(17)*u(8)*u(12)*u(2)*u(14)*u(6)-u(17)^2*u(8)*u(12)*u(2)*u(9)-u(17)*u(8)*u(15)*u(5)*u(11)*u(3)-u(17)^2*u(8)*u(15)*u(5)*u(9)-u(17)*u(8)^2*u(18)*u(11)*u(3)-u(17)*u(8)^2*u(18)*u(14)*u(6)-u(10)^2*u(2)*u(14)*u(4)*u(1)-u(10)*u(2)*u(14)*u(4)*u(17)*u(8)-u(10)*u(2)*u(14)*u(4)*u(16)*u(7)-u(10)*u(2)^2*u(17)*u(7)*u(11)-u(10)^2*u(2)*u(17)*u(7)*u(1)-u(10)*u(2)*u(17)*u(7)*u(14)*u(5)-u(10)*u(2)*u(17)*u(7)*u(13)*u(4)-u(10)*u(2)*u(12)*u(1)*u(14)*u(6)-u(10)*u(2)*u(12)*u(1)*u(17)*u(9)-u(10)*u(2)*u(15)*u(4)*u(11)*u(3)-u(10)*u(2)*u(15)*u(4)*u(14)*u(6)-u(10)*u(2)*u(15)*u(4)*u(17)*u(9)-u(10)*u(2)*u(18)*u(7)*u(11)*u(3)-u(10)*u(2)*u(18)*u(7)*u(14)*u(6)-u(10)*u(2)*u(18)*u(7)*u(17)*u(9)-u(13)*u(5)*u(11)^2*u(1)*u(2)-u(13)*u(5)*u(11)*u(1)^2*u(10)-u(13)*u(5)*u(17)*u(7)^2*u(16)-u(13)*u(5)*u(17)^2*u(7)*u(8)-u(13)*u(5)^2*u(11)*u(1)*u(14)-u(13)^2*u(5)*u(11)*u(1)*u(4)-u(13)*u(5)*u(11)*u(1)*u(17)*u(8)-u(13)*u(5)*u(11)*u(1)*u(16)*u(7)-u(13)*u(5)*u(17)*u(7)*u(11)*u(2)-u(13)*u(5)*u(17)*u(7)*u(10)*u(1)-u(13)*u(5)^2*u(17)*u(7)*u(14)-u(13)^2*u(5)*u(17)*u(7)*u(4)-u(13)*u(5)*u(12)*u(1)*u(11)*u(3)-u(13)*u(5)*u(12)*u(1)*u(14)*u(6)-u(13)*u(5)*u(12)*u(1)*u(17)*u(9)-u(13)*u(5)*u(15)*u(4)*u(11)*u(3)-u(13)*u(5)*u(15)*u(4)*u(17)*u(9)-u(13)*u(5)*u(18)*u(7)*u(11)*u(3)-u(13)*u(5)*u(18)*u(7)*u(14)*u(6)-u(13)*u(5)*u(18)*u(7)*u(17)*u(9)-u(16)*u(8)*u(14)^2*u(4)*u(5)-u(16)*u(8)*u(11)^2*u(1)*u(2)-u(16)*u(8)*u(14)*u(4)^2*u(13)-u(16)*u(8)*u(11)*u(1)^2*u(10)-u(16)*u(8)*u(11)*u(1)*u(14)*u(5)-u(16)*u(8)*u(11)*u(1)*u(13)*u(4)-u(16)*u(8)^2*u(11)*u(1)*u(17)-u(16)^2*u(8)*u(11)*u(1)*u(7)-u(16)*u(8)*u(14)*u(4)*u(11)*u(2)-u(16)*u(8)*u(14)*u(4)*u(10)*u(1)-u(16)*u(8)^2*u(14)*u(4)*u(17)-u(16)^2*u(8)*u(14)*u(4)*u(7)-u(16)*u(8)*u(12)*u(1)*u(11)*u(3)-u(16)*u(8)*u(12)*u(1)*u(14)*u(6)-u(16)*u(8)*u(12)*u(1)*u(17)*u(9)-u(16)*u(8)*u(15)*u(4)*u(11)*u(3)-u(16)*u(8)*u(15)*u(4)*u(14)*u(6)-u(16)*u(8)*u(15)*u(4)*u(17)*u(9)-u(16)*u(8)*u(18)*u(7)*u(11)*u(3)-u(16)*u(8)*u(18)*u(7)*u(14)*u(6)-u(10)*u(3)*u(15)^2*u(4)*u(6)-u(10)*u(3)*u(15)*u(4)^2*u(13)-u(10)*u(3)*u(18)^2*u(7)*u(9)-u(10)*u(3)*u(18)*u(7)^2*u(16)-u(10)*u(3)*u(11)*u(1)*u(15)*u(5)-u(10)*u(3)*u(11)*u(1)*u(18)*u(8)-u(10)*u(3)*u(14)*u(4)*u(12)*u(2)-u(10)*u(3)*u(14)*u(4)*u(15)*u(5)-u(10)*u(3)*u(14)*u(4)*u(18)*u(8)-u(10)*u(3)*u(17)*u(7)*u(12)*u(2)-u(10)*u(3)*u(17)*u(7)*u(15)*u(5)-u(10)*u(3)*u(17)*u(7)*u(18)*u(8)-u(10)*u(3)^2*u(15)*u(4)*u(12)-u(10)^2*u(3)*u(15)*u(4)*u(1)-u(10)*u(3)*u(15)*u(4)*u(18)*u(9)-u(10)*u(3)*u(15)*u(4)*u(16)*u(7)-u(10)*u(3)^2*u(18)*u(7)*u(12)-u(10)^2*u(3)*u(18)*u(7)*u(1)-u(10)*u(3)*u(18)*u(7)*u(15)*u(6)-u(10)*u(3)*u(18)*u(7)*u(13)*u(4)-u(13)*u(6)*u(12)*u(1)^2*u(10)-u(13)*u(6)*u(12)^2*u(1)*u(3)-u(13)*u(6)*u(18)^2*u(7)*u(9)-u(13)*u(6)*u(18)*u(7)^2*u(16)-u(13)*u(6)*u(11)*u(1)*u(12)*u(2)-u(13)*u(6)*u(11)*u(1)*u(15)*u(5)-u(13)*u(6)*u(11)*u(1)*u(18)*u(8)-u(13)*u(6)*u(14)*u(4)*u(12)*u(2)-u(13)*u(6)*u(14)*u(4)*u(18)*u(8)-u(13)*u(6)*u(17)*u(7)*u(12)*u(2)-u(13)*u(6)*u(17)*u(7)*u(15)*u(5)-u(13)*u(6)*u(17)*u(7)*u(18)*u(8)-u(13)*u(6)^2*u(12)*u(1)*u(15)-u(13)^2*u(6)*u(12)*u(1)*u(4)-u(13)*u(6)*u(12)*u(1)*u(18)*u(9)-u(13)*u(6)*u(12)*u(1)*u(16)*u(7)-u(13)*u(6)*u(18)*u(7)*u(12)*u(3)-u(13)*u(6)*u(18)*u(7)*u(10)*u(1)-u(13)*u(6)^2*u(18)*u(7)*u(15)-u(13)^2*u(6)*u(18)*u(7)*u(4)-u(16)*u(9)*u(12)*u(1)^2*u(10)-u(16)*u(9)*u(12)^2*u(1)*u(3)-u(16)*u(9)*u(15)^2*u(4)*u(6)-u(16)*u(9)*u(15)*u(4)^2*u(13)-u(16)*u(9)*u(11)*u(1)*u(12)*u(2)-u(16)*u(9)*u(11)*u(1)*u(15)*u(5)-u(16)*u(9)*u(11)*u(1)*u(18)*u(8)-u(16)*u(9)*u(14)*u(4)*u(12)*u(2)-u(16)*u(9)*u(14)*u(4)*u(15)*u(5)-u(16)*u(9)*u(14)*u(4)*u(18)*u(8)-u(16)*u(9)*u(17)*u(7)*u(12)*u(2)-u(16)*u(9)*u(17)*u(7)*u(15)*u(5)-u(16)*u(9)*u(12)*u(1)*u(15)*u(6)-u(16)*u(9)*u(12)*u(1)*u(13)*u(4)-u(16)*u(9)^2*u(12)*u(1)*u(18)-u(16)^2*u(9)*u(12)*u(1)*u(7)-u(16)*u(9)*u(15)*u(4)*u(12)*u(3)-u(16)*u(9)*u(15)*u(4)*u(10)*u(1)-u(16)*u(9)^2*u(15)*u(4)*u(18)-u(16)^2*u(9)*u(15)*u(4)*u(7))*u(21)
  invL2 : Fcn  Expr=2*(u(13)^2*u(5)*u(4)+u(16)^2*u(8)*u(7)+u(10)*u(2)^2*u(11)+u(16)*u(8)^2*u(17)+u(13)*u(5)^2*u(14)+u(10)^2*u(2)*u(1)+u(10)*u(2)*u(14)*u(5)+u(10)*u(2)*u(13)*u(4)+u(10)*u(2)*u(17)*u(8)+u(10)*u(2)*u(16)*u(7)+u(13)*u(5)*u(11)*u(2)+u(13)*u(5)*u(10)*u(1)+u(13)*u(5)*u(17)*u(8)+u(13)*u(5)*u(16)*u(7)+u(16)*u(8)*u(11)*u(2)+u(16)*u(8)*u(10)*u(1)+u(16)*u(8)*u(14)*u(5)+u(16)*u(8)*u(13)*u(4)+u(12)*u(2)*u(10)*u(3)+u(12)*u(2)*u(13)*u(6)+u(12)*u(2)*u(16)*u(9)+u(15)*u(5)*u(10)*u(3)+u(15)*u(5)*u(13)*u(6)+u(15)*u(5)*u(16)*u(9)+u(18)*u(8)*u(10)*u(3)+u(18)*u(8)*u(13)*u(6)+u(18)*u(8)*u(16)*u(9))/(u(12)*u(3)*u(13)^2*u(4)^2+u(12)*u(3)*u(16)^2*u(7)^2+u(12)^2*u(3)^2*u(14)*u(5)+u(12)^2*u(3)^2*u(13)*u(4)+u(12)^2*u(3)^2*u(17)*u(8)+u(12)^2*u(3)^2*u(16)*u(7)+u(11)*u(2)*u(13)^2*u(4)^2+u(11)*u(2)*u(16)^2*u(7)^2+u(11)^2*u(2)^2*u(15)*u(6)+u(11)^2*u(2)^2*u(13)*u(4)+u(11)^2*u(2)^2*u(18)*u(9)+u(11)^2*u(2)^2*u(16)*u(7)+u(15)*u(6)*u(10)^2*u(1)^2+u(15)*u(6)*u(16)^2*u(7)^2+u(15)^2*u(6)^2*u(11)*u(2)+u(15)^2*u(6)^2*u(10)*u(1)+u(15)^2*u(6)^2*u(17)*u(8)+u(15)^2*u(6)^2*u(16)*u(7)+u(14)*u(5)*u(10)^2*u(1)^2+u(14)*u(5)*u(16)^2*u(7)^2+u(14)^2*u(5)^2*u(12)*u(3)+u(14)^2*u(5)^2*u(10)*u(1)+u(14)^2*u(5)^2*u(18)*u(9)+u(14)^2*u(5)^2*u(16)*u(7)+u(18)*u(9)*u(10)^2*u(1)^2+u(18)*u(9)*u(13)^2*u(4)^2+u(18)^2*u(9)^2*u(11)*u(2)+u(18)^2*u(9)^2*u(10)*u(1)+u(18)^2*u(9)^2*u(14)*u(5)+u(18)^2*u(9)^2*u(13)*u(4)+u(17)*u(8)*u(10)^2*u(1)^2+u(17)*u(8)*u(13)^2*u(4)^2+u(17)^2*u(8)^2*u(12)*u(3)+u(17)^2*u(8)^2*u(10)*u(1)+u(17)^2*u(8)^2*u(15)*u(6)+u(17)^2*u(8)^2*u(13)*u(4)-u(10)*u(2)*u(14)^2*u(4)*u(5)-u(10)*u(2)*u(14)*u(4)^2*u(13)-u(10)*u(2)*u(17)*u(7)^2*u(16)-u(10)*u(2)*u(17)^2*u(7)*u(8)-u(10)*u(2)^2*u(14)*u(4)*u(11)+2*u(12)*u(3)*u(10)*u(1)*u(14)*u(5)+u(12)*u(3)*u(10)*u(1)*u(13)*u(4)+2*u(12)*u(3)*u(10)*u(1)*u(17)*u(8)+u(12)*u(3)*u(10)*u(1)*u(16)*u(7)+u(12)*u(3)*u(15)*u(6)*u(11)*u(2)+u(12)*u(3)*u(15)*u(6)*u(10)*u(1)+u(12)*u(3)*u(15)*u(6)*u(13)*u(4)+2*u(12)*u(3)*u(15)*u(6)*u(17)*u(8)+2*u(12)*u(3)*u(15)*u(6)*u(16)*u(7)+2*u(12)*u(3)*u(13)*u(4)*u(11)*u(2)+2*u(12)*u(3)*u(13)*u(4)*u(14)*u(5)+2*u(12)*u(3)*u(13)*u(4)*u(17)*u(8)+2*u(12)*u(3)*u(13)*u(4)*u(16)*u(7)+u(12)*u(3)*u(18)*u(9)*u(11)*u(2)+u(12)*u(3)*u(18)*u(9)*u(10)*u(1)+2*u(12)*u(3)*u(18)*u(9)*u(14)*u(5)+2*u(12)*u(3)*u(18)*u(9)*u(13)*u(4)+u(12)*u(3)*u(18)*u(9)*u(16)*u(7)+2*u(12)*u(3)*u(16)*u(7)*u(11)*u(2)+2*u(12)*u(3)*u(16)*u(7)*u(14)*u(5)+2*u(12)*u(3)*u(16)*u(7)*u(17)*u(8)-u(12)^2*u(3)*u(2)*u(14)*u(6)-u(12)^2*u(3)*u(2)*u(17)*u(9)-u(12)*u(3)^2*u(15)*u(5)*u(11)-u(12)*u(3)*u(15)*u(5)*u(17)*u(9)-u(12)*u(3)^2*u(18)*u(8)*u(11)-u(12)*u(3)*u(18)*u(8)*u(14)*u(6)+u(11)*u(2)*u(12)*u(3)*u(14)*u(5)+u(11)*u(2)*u(12)*u(3)*u(17)*u(8)+u(11)*u(2)*u(10)*u(1)*u(14)*u(5)+u(11)*u(2)*u(10)*u(1)*u(13)*u(4)+u(11)*u(2)*u(10)*u(1)*u(17)*u(8)+u(11)*u(2)*u(10)*u(1)*u(16)*u(7)+2*u(11)*u(2)*u(15)*u(6)*u(10)*u(1)+2*u(11)*u(2)*u(15)*u(6)*u(13)*u(4)+2*u(11)*u(2)*u(15)*u(6)*u(17)*u(8)+2*u(11)*u(2)*u(15)*u(6)*u(16)*u(7)+u(11)*u(2)*u(13)*u(4)*u(14)*u(5)+2*u(11)*u(2)*u(13)*u(4)*u(17)*u(8)+2*u(11)*u(2)*u(13)*u(4)*u(16)*u(7)+2*u(11)*u(2)*u(18)*u(9)*u(10)*u(1)+2*u(11)*u(2)*u(18)*u(9)*u(14)*u(5)+2*u(11)*u(2)*u(18)*u(9)*u(13)*u(4)+2*u(11)*u(2)*u(18)*u(9)*u(16)*u(7)+2*u(11)*u(2)*u(16)*u(7)*u(14)*u(5)+u(11)*u(2)*u(16)*u(7)*u(17)*u(8)-u(11)*u(2)^2*u(12)*u(14)*u(6)-u(11)*u(2)^2*u(12)*u(17)*u(9)-u(11)^2*u(2)*u(15)*u(5)*u(3)-u(11)*u(2)*u(15)*u(5)*u(17)*u(9)-u(11)^2*u(2)*u(18)*u(8)*u(3)-u(11)*u(2)*u(18)*u(8)*u(14)*u(6)+u(15)*u(6)*u(12)*u(3)*u(14)*u(5)+2*u(15)*u(6)*u(10)*u(1)*u(14)*u(5)+u(15)*u(6)*u(10)*u(1)*u(13)*u(4)+2*u(15)*u(6)*u(10)*u(1)*u(17)*u(8)+2*u(15)*u(6)*u(10)*u(1)*u(16)*u(7)+2*u(15)*u(6)*u(13)*u(4)*u(17)*u(8)+u(15)*u(6)*u(13)*u(4)*u(16)*u(7)+2*u(15)*u(6)*u(18)*u(9)*u(11)*u(2)+2*u(15)*u(6)*u(18)*u(9)*u(10)*u(1)+u(15)*u(6)*u(18)*u(9)*u(14)*u(5)+u(15)*u(6)*u(18)*u(9)*u(13)*u(4)+u(15)*u(6)*u(18)*u(9)*u(16)*u(7)+2*u(15)*u(6)*u(16)*u(7)*u(14)*u(5)+2*u(15)*u(6)*u(16)*u(7)*u(17)*u(8)-u(15)*u(6)^2*u(12)*u(2)*u(14)-u(15)*u(6)*u(12)*u(2)*u(17)*u(9)-u(15)^2*u(6)*u(5)*u(11)*u(3)-u(15)^2*u(6)*u(5)*u(17)*u(9)-u(15)*u(6)*u(18)*u(8)*u(11)*u(3)-u(15)*u(6)^2*u(18)*u(8)*u(14)+2*u(14)*u(5)*u(12)*u(3)*u(17)*u(8)+u(14)*u(5)*u(10)*u(1)*u(13)*u(4)+2*u(14)*u(5)*u(10)*u(1)*u(17)*u(8)+2*u(14)*u(5)*u(10)*u(1)*u(16)*u(7)+u(14)*u(5)*u(15)*u(6)*u(11)*u(2)+u(14)*u(5)*u(15)*u(6)*u(17)*u(8)+u(14)*u(5)*u(13)*u(4)*u(17)*u(8)+u(14)*u(5)*u(13)*u(4)*u(16)*u(7)+2*u(14)*u(5)*u(18)*u(9)*u(10)*u(1)+2*u(14)*u(5)*u(18)*u(9)*u(13)*u(4)+2*u(14)*u(5)*u(18)*u(9)*u(16)*u(7)+u(14)*u(5)*u(16)*u(7)*u(17)*u(8)-u(14)^2*u(5)*u(12)*u(2)*u(6)-u(14)*u(5)*u(12)*u(2)*u(17)*u(9)-u(14)*u(5)^2*u(15)*u(11)*u(3)-u(14)*u(5)^2*u(15)*u(17)*u(9)-u(14)*u(5)*u(18)*u(8)*u(11)*u(3)-u(14)^2*u(5)*u(18)*u(8)*u(6)+u(18)*u(9)*u(12)*u(3)*u(17)*u(8)+2*u(18)*u(9)*u(10)*u(1)*u(13)*u(4)+2*u(18)*u(9)*u(10)*u(1)*u(17)*u(8)+u(18)*u(9)*u(10)*u(1)*u(16)*u(7)+u(18)*u(9)*u(15)*u(6)*u(17)*u(8)+2*u(18)*u(9)*u(13)*u(4)*u(17)*u(8)+u(18)*u(9)*u(13)*u(4)*u(16)*u(7)-u(18)*u(9)*u(12)*u(2)*u(14)*u(6)-u(18)*u(9)^2*u(12)*u(2)*u(17)-u(18)*u(9)*u(15)*u(5)*u(11)*u(3)-u(18)*u(9)^2*u(15)*u(5)*u(17)-u(18)^2*u(9)*u(8)*u(11)*u(3)-u(18)^2*u(9)*u(8)*u(14)*u(6)+2*u(17)*u(8)*u(10)*u(1)*u(13)*u(4)+u(17)*u(8)*u(10)*u(1)*u(16)*u(7)+u(17)*u(8)*u(13)*u(4)*u(16)*u(7)+u(17)*u(8)*u(18)*u(9)*u(11)*u(2)+u(17)*u(8)*u(18)*u(9)*u(14)*u(5)-u(17)*u(8)*u(12)*u(2)*u(14)*u(6)-u(17)^2*u(8)*u(12)*u(2)*u(9)-u(17)*u(8)*u(15)*u(5)*u(11)*u(3)-u(17)^2*u(8)*u(15)*u(5)*u(9)-u(17)*u(8)^2*u(18)*u(11)*u(3)-u(17)*u(8)^2*u(18)*u(14)*u(6)-u(10)^2*u(2)*u(14)*u(4)*u(1)-u(10)*u(2)*u(14)*u(4)*u(17)*u(8)-u(10)*u(2)*u(14)*u(4)*u(16)*u(7)-u(10)*u(2)^2*u(17)*u(7)*u(11)-u(10)^2*u(2)*u(17)*u(7)*u(1)-u(10)*u(2)*u(17)*u(7)*u(14)*u(5)-u(10)*u(2)*u(17)*u(7)*u(13)*u(4)-u(10)*u(2)*u(12)*u(1)*u(14)*u(6)-u(10)*u(2)*u(12)*u(1)*u(17)*u(9)-u(10)*u(2)*u(15)*u(4)*u(11)*u(3)-u(10)*u(2)*u(15)*u(4)*u(14)*u(6)-u(10)*u(2)*u(15)*u(4)*u(17)*u(9)-u(10)*u(2)*u(18)*u(7)*u(11)*u(3)-u(10)*u(2)*u(18)*u(7)*u(14)*u(6)-u(10)*u(2)*u(18)*u(7)*u(17)*u(9)-u(13)*u(5)*u(11)^2*u(1)*u(2)-u(13)*u(5)*u(11)*u(1)^2*u(10)-u(13)*u(5)*u(17)*u(7)^2*u(16)-u(13)*u(5)*u(17)^2*u(7)*u(8)-u(13)*u(5)^2*u(11)*u(1)*u(14)-u(13)^2*u(5)*u(11)*u(1)*u(4)-u(13)*u(5)*u(11)*u(1)*u(17)*u(8)-u(13)*u(5)*u(11)*u(1)*u(16)*u(7)-u(13)*u(5)*u(17)*u(7)*u(11)*u(2)-u(13)*u(5)*u(17)*u(7)*u(10)*u(1)-u(13)*u(5)^2*u(17)*u(7)*u(14)-u(13)^2*u(5)*u(17)*u(7)*u(4)-u(13)*u(5)*u(12)*u(1)*u(11)*u(3)-u(13)*u(5)*u(12)*u(1)*u(14)*u(6)-u(13)*u(5)*u(12)*u(1)*u(17)*u(9)-u(13)*u(5)*u(15)*u(4)*u(11)*u(3)-u(13)*u(5)*u(15)*u(4)*u(17)*u(9)-u(13)*u(5)*u(18)*u(7)*u(11)*u(3)-u(13)*u(5)*u(18)*u(7)*u(14)*u(6)-u(13)*u(5)*u(18)*u(7)*u(17)*u(9)-u(16)*u(8)*u(14)^2*u(4)*u(5)-u(16)*u(8)*u(11)^2*u(1)*u(2)-u(16)*u(8)*u(14)*u(4)^2*u(13)-u(16)*u(8)*u(11)*u(1)^2*u(10)-u(16)*u(8)*u(11)*u(1)*u(14)*u(5)-u(16)*u(8)*u(11)*u(1)*u(13)*u(4)-u(16)*u(8)^2*u(11)*u(1)*u(17)-u(16)^2*u(8)*u(11)*u(1)*u(7)-u(16)*u(8)*u(14)*u(4)*u(11)*u(2)-u(16)*u(8)*u(14)*u(4)*u(10)*u(1)-u(16)*u(8)^2*u(14)*u(4)*u(17)-u(16)^2*u(8)*u(14)*u(4)*u(7)-u(16)*u(8)*u(12)*u(1)*u(11)*u(3)-u(16)*u(8)*u(12)*u(1)*u(14)*u(6)-u(16)*u(8)*u(12)*u(1)*u(17)*u(9)-u(16)*u(8)*u(15)*u(4)*u(11)*u(3)-u(16)*u(8)*u(15)*u(4)*u(14)*u(6)-u(16)*u(8)*u(15)*u(4)*u(17)*u(9)-u(16)*u(8)*u(18)*u(7)*u(11)*u(3)-u(16)*u(8)*u(18)*u(7)*u(14)*u(6)-u(10)*u(3)*u(15)^2*u(4)*u(6)-u(10)*u(3)*u(15)*u(4)^2*u(13)-u(10)*u(3)*u(18)^2*u(7)*u(9)-u(10)*u(3)*u(18)*u(7)^2*u(16)-u(10)*u(3)*u(11)*u(1)*u(15)*u(5)-u(10)*u(3)*u(11)*u(1)*u(18)*u(8)-u(10)*u(3)*u(14)*u(4)*u(12)*u(2)-u(10)*u(3)*u(14)*u(4)*u(15)*u(5)-u(10)*u(3)*u(14)*u(4)*u(18)*u(8)-u(10)*u(3)*u(17)*u(7)*u(12)*u(2)-u(10)*u(3)*u(17)*u(7)*u(15)*u(5)-u(10)*u(3)*u(17)*u(7)*u(18)*u(8)-u(10)*u(3)^2*u(15)*u(4)*u(12)-u(10)^2*u(3)*u(15)*u(4)*u(1)-u(10)*u(3)*u(15)*u(4)*u(18)*u(9)-u(10)*u(3)*u(15)*u(4)*u(16)*u(7)-u(10)*u(3)^2*u(18)*u(7)*u(12)-u(10)^2*u(3)*u(18)*u(7)*u(1)-u(10)*u(3)*u(18)*u(7)*u(15)*u(6)-u(10)*u(3)*u(18)*u(7)*u(13)*u(4)-u(13)*u(6)*u(12)*u(1)^2*u(10)-u(13)*u(6)*u(12)^2*u(1)*u(3)-u(13)*u(6)*u(18)^2*u(7)*u(9)-u(13)*u(6)*u(18)*u(7)^2*u(16)-u(13)*u(6)*u(11)*u(1)*u(12)*u(2)-u(13)*u(6)*u(11)*u(1)*u(15)*u(5)-u(13)*u(6)*u(11)*u(1)*u(18)*u(8)-u(13)*u(6)*u(14)*u(4)*u(12)*u(2)-u(13)*u(6)*u(14)*u(4)*u(18)*u(8)-u(13)*u(6)*u(17)*u(7)*u(12)*u(2)-u(13)*u(6)*u(17)*u(7)*u(15)*u(5)-u(13)*u(6)*u(17)*u(7)*u(18)*u(8)-u(13)*u(6)^2*u(12)*u(1)*u(15)-u(13)^2*u(6)*u(12)*u(1)*u(4)-u(13)*u(6)*u(12)*u(1)*u(18)*u(9)-u(13)*u(6)*u(12)*u(1)*u(16)*u(7)-u(13)*u(6)*u(18)*u(7)*u(12)*u(3)-u(13)*u(6)*u(18)*u(7)*u(10)*u(1)-u(13)*u(6)^2*u(18)*u(7)*u(15)-u(13)^2*u(6)*u(18)*u(7)*u(4)-u(16)*u(9)*u(12)*u(1)^2*u(10)-u(16)*u(9)*u(12)^2*u(1)*u(3)-u(16)*u(9)*u(15)^2*u(4)*u(6)-u(16)*u(9)*u(15)*u(4)^2*u(13)-u(16)*u(9)*u(11)*u(1)*u(12)*u(2)-u(16)*u(9)*u(11)*u(1)*u(15)*u(5)-u(16)*u(9)*u(11)*u(1)*u(18)*u(8)-u(16)*u(9)*u(14)*u(4)*u(12)*u(2)-u(16)*u(9)*u(14)*u(4)*u(15)*u(5)-u(16)*u(9)*u(14)*u(4)*u(18)*u(8)-u(16)*u(9)*u(17)*u(7)*u(12)*u(2)-u(16)*u(9)*u(17)*u(7)*u(15)*u(5)-u(16)*u(9)*u(12)*u(1)*u(15)*u(6)-u(16)*u(9)*u(12)*u(1)*u(13)*u(4)-u(16)*u(9)^2*u(12)*u(1)*u(18)-u(16)^2*u(9)*u(12)*u(1)*u(7)-u(16)*u(9)*u(15)*u(4)*u(12)*u(3)-u(16)*u(9)*u(15)*u(4)*u(10)*u(1)-u(16)*u(9)^2*u(15)*u(4)*u(18)-u(16)^2*u(9)*u(15)*u(4)*u(7))*u(19)+2*(u(12)*u(3)*u(11)*u(2)+u(12)*u(3)*u(14)*u(5)+u(12)*u(3)*u(13)*u(4)+u(12)*u(3)*u(17)*u(8)+u(12)*u(3)*u(16)*u(7)+u(10)*u(1)*u(11)*u(2)+u(10)*u(1)*u(14)*u(5)+u(10)*u(1)*u(17)*u(8)+u(15)*u(6)*u(11)*u(2)+u(15)*u(6)*u(10)*u(1)+u(15)*u(6)*u(14)*u(5)+u(15)*u(6)*u(17)*u(8)+u(15)*u(6)*u(16)*u(7)+u(13)*u(4)*u(11)*u(2)+u(13)*u(4)*u(14)*u(5)+u(13)*u(4)*u(17)*u(8)+u(18)*u(9)*u(11)*u(2)+u(18)*u(9)*u(10)*u(1)+u(18)*u(9)*u(14)*u(5)+u(18)*u(9)*u(13)*u(4)+u(18)*u(9)*u(17)*u(8)+u(16)*u(7)*u(11)*u(2)+u(16)*u(7)*u(14)*u(5)+u(16)*u(7)*u(17)*u(8)+u(11)^2*u(2)^2+u(14)^2*u(5)^2+u(17)^2*u(8)^2+2*u(11)*u(2)*u(14)*u(5)+2*u(11)*u(2)*u(17)*u(8)+2*u(14)*u(5)*u(17)*u(8)-u(12)*u(1)*u(13)*u(6)-u(12)*u(1)*u(16)*u(9)-u(15)*u(4)*u(10)*u(3)-u(15)*u(4)*u(16)*u(9)-u(18)*u(7)*u(10)*u(3)-u(18)*u(7)*u(13)*u(6))/(u(12)*u(3)*u(13)^2*u(4)^2+u(12)*u(3)*u(16)^2*u(7)^2+u(12)^2*u(3)^2*u(14)*u(5)+u(12)^2*u(3)^2*u(13)*u(4)+u(12)^2*u(3)^2*u(17)*u(8)+u(12)^2*u(3)^2*u(16)*u(7)+u(11)*u(2)*u(13)^2*u(4)^2+u(11)*u(2)*u(16)^2*u(7)^2+u(11)^2*u(2)^2*u(15)*u(6)+u(11)^2*u(2)^2*u(13)*u(4)+u(11)^2*u(2)^2*u(18)*u(9)+u(11)^2*u(2)^2*u(16)*u(7)+u(15)*u(6)*u(10)^2*u(1)^2+u(15)*u(6)*u(16)^2*u(7)^2+u(15)^2*u(6)^2*u(11)*u(2)+u(15)^2*u(6)^2*u(10)*u(1)+u(15)^2*u(6)^2*u(17)*u(8)+u(15)^2*u(6)^2*u(16)*u(7)+u(14)*u(5)*u(10)^2*u(1)^2+u(14)*u(5)*u(16)^2*u(7)^2+u(14)^2*u(5)^2*u(12)*u(3)+u(14)^2*u(5)^2*u(10)*u(1)+u(14)^2*u(5)^2*u(18)*u(9)+u(14)^2*u(5)^2*u(16)*u(7)+u(18)*u(9)*u(10)^2*u(1)^2+u(18)*u(9)*u(13)^2*u(4)^2+u(18)^2*u(9)^2*u(11)*u(2)+u(18)^2*u(9)^2*u(10)*u(1)+u(18)^2*u(9)^2*u(14)*u(5)+u(18)^2*u(9)^2*u(13)*u(4)+u(17)*u(8)*u(10)^2*u(1)^2+u(17)*u(8)*u(13)^2*u(4)^2+u(17)^2*u(8)^2*u(12)*u(3)+u(17)^2*u(8)^2*u(10)*u(1)+u(17)^2*u(8)^2*u(15)*u(6)+u(17)^2*u(8)^2*u(13)*u(4)-u(10)*u(2)*u(14)^2*u(4)*u(5)-u(10)*u(2)*u(14)*u(4)^2*u(13)-u(10)*u(2)*u(17)*u(7)^2*u(16)-u(10)*u(2)*u(17)^2*u(7)*u(8)-u(10)*u(2)^2*u(14)*u(4)*u(11)+2*u(12)*u(3)*u(10)*u(1)*u(14)*u(5)+u(12)*u(3)*u(10)*u(1)*u(13)*u(4)+2*u(12)*u(3)*u(10)*u(1)*u(17)*u(8)+u(12)*u(3)*u(10)*u(1)*u(16)*u(7)+u(12)*u(3)*u(15)*u(6)*u(11)*u(2)+u(12)*u(3)*u(15)*u(6)*u(10)*u(1)+u(12)*u(3)*u(15)*u(6)*u(13)*u(4)+2*u(12)*u(3)*u(15)*u(6)*u(17)*u(8)+2*u(12)*u(3)*u(15)*u(6)*u(16)*u(7)+2*u(12)*u(3)*u(13)*u(4)*u(11)*u(2)+2*u(12)*u(3)*u(13)*u(4)*u(14)*u(5)+2*u(12)*u(3)*u(13)*u(4)*u(17)*u(8)+2*u(12)*u(3)*u(13)*u(4)*u(16)*u(7)+u(12)*u(3)*u(18)*u(9)*u(11)*u(2)+u(12)*u(3)*u(18)*u(9)*u(10)*u(1)+2*u(12)*u(3)*u(18)*u(9)*u(14)*u(5)+2*u(12)*u(3)*u(18)*u(9)*u(13)*u(4)+u(12)*u(3)*u(18)*u(9)*u(16)*u(7)+2*u(12)*u(3)*u(16)*u(7)*u(11)*u(2)+2*u(12)*u(3)*u(16)*u(7)*u(14)*u(5)+2*u(12)*u(3)*u(16)*u(7)*u(17)*u(8)-u(12)^2*u(3)*u(2)*u(14)*u(6)-u(12)^2*u(3)*u(2)*u(17)*u(9)-u(12)*u(3)^2*u(15)*u(5)*u(11)-u(12)*u(3)*u(15)*u(5)*u(17)*u(9)-u(12)*u(3)^2*u(18)*u(8)*u(11)-u(12)*u(3)*u(18)*u(8)*u(14)*u(6)+u(11)*u(2)*u(12)*u(3)*u(14)*u(5)+u(11)*u(2)*u(12)*u(3)*u(17)*u(8)+u(11)*u(2)*u(10)*u(1)*u(14)*u(5)+u(11)*u(2)*u(10)*u(1)*u(13)*u(4)+u(11)*u(2)*u(10)*u(1)*u(17)*u(8)+u(11)*u(2)*u(10)*u(1)*u(16)*u(7)+2*u(11)*u(2)*u(15)*u(6)*u(10)*u(1)+2*u(11)*u(2)*u(15)*u(6)*u(13)*u(4)+2*u(11)*u(2)*u(15)*u(6)*u(17)*u(8)+2*u(11)*u(2)*u(15)*u(6)*u(16)*u(7)+u(11)*u(2)*u(13)*u(4)*u(14)*u(5)+2*u(11)*u(2)*u(13)*u(4)*u(17)*u(8)+2*u(11)*u(2)*u(13)*u(4)*u(16)*u(7)+2*u(11)*u(2)*u(18)*u(9)*u(10)*u(1)+2*u(11)*u(2)*u(18)*u(9)*u(14)*u(5)+2*u(11)*u(2)*u(18)*u(9)*u(13)*u(4)+2*u(11)*u(2)*u(18)*u(9)*u(16)*u(7)+2*u(11)*u(2)*u(16)*u(7)*u(14)*u(5)+u(11)*u(2)*u(16)*u(7)*u(17)*u(8)-u(11)*u(2)^2*u(12)*u(14)*u(6)-u(11)*u(2)^2*u(12)*u(17)*u(9)-u(11)^2*u(2)*u(15)*u(5)*u(3)-u(11)*u(2)*u(15)*u(5)*u(17)*u(9)-u(11)^2*u(2)*u(18)*u(8)*u(3)-u(11)*u(2)*u(18)*u(8)*u(14)*u(6)+u(15)*u(6)*u(12)*u(3)*u(14)*u(5)+2*u(15)*u(6)*u(10)*u(1)*u(14)*u(5)+u(15)*u(6)*u(10)*u(1)*u(13)*u(4)+2*u(15)*u(6)*u(10)*u(1)*u(17)*u(8)+2*u(15)*u(6)*u(10)*u(1)*u(16)*u(7)+2*u(15)*u(6)*u(13)*u(4)*u(17)*u(8)+u(15)*u(6)*u(13)*u(4)*u(16)*u(7)+2*u(15)*u(6)*u(18)*u(9)*u(11)*u(2)+2*u(15)*u(6)*u(18)*u(9)*u(10)*u(1)+u(15)*u(6)*u(18)*u(9)*u(14)*u(5)+u(15)*u(6)*u(18)*u(9)*u(13)*u(4)+u(15)*u(6)*u(18)*u(9)*u(16)*u(7)+2*u(15)*u(6)*u(16)*u(7)*u(14)*u(5)+2*u(15)*u(6)*u(16)*u(7)*u(17)*u(8)-u(15)*u(6)^2*u(12)*u(2)*u(14)-u(15)*u(6)*u(12)*u(2)*u(17)*u(9)-u(15)^2*u(6)*u(5)*u(11)*u(3)-u(15)^2*u(6)*u(5)*u(17)*u(9)-u(15)*u(6)*u(18)*u(8)*u(11)*u(3)-u(15)*u(6)^2*u(18)*u(8)*u(14)+2*u(14)*u(5)*u(12)*u(3)*u(17)*u(8)+u(14)*u(5)*u(10)*u(1)*u(13)*u(4)+2*u(14)*u(5)*u(10)*u(1)*u(17)*u(8)+2*u(14)*u(5)*u(10)*u(1)*u(16)*u(7)+u(14)*u(5)*u(15)*u(6)*u(11)*u(2)+u(14)*u(5)*u(15)*u(6)*u(17)*u(8)+u(14)*u(5)*u(13)*u(4)*u(17)*u(8)+u(14)*u(5)*u(13)*u(4)*u(16)*u(7)+2*u(14)*u(5)*u(18)*u(9)*u(10)*u(1)+2*u(14)*u(5)*u(18)*u(9)*u(13)*u(4)+2*u(14)*u(5)*u(18)*u(9)*u(16)*u(7)+u(14)*u(5)*u(16)*u(7)*u(17)*u(8)-u(14)^2*u(5)*u(12)*u(2)*u(6)-u(14)*u(5)*u(12)*u(2)*u(17)*u(9)-u(14)*u(5)^2*u(15)*u(11)*u(3)-u(14)*u(5)^2*u(15)*u(17)*u(9)-u(14)*u(5)*u(18)*u(8)*u(11)*u(3)-u(14)^2*u(5)*u(18)*u(8)*u(6)+u(18)*u(9)*u(12)*u(3)*u(17)*u(8)+2*u(18)*u(9)*u(10)*u(1)*u(13)*u(4)+2*u(18)*u(9)*u(10)*u(1)*u(17)*u(8)+u(18)*u(9)*u(10)*u(1)*u(16)*u(7)+u(18)*u(9)*u(15)*u(6)*u(17)*u(8)+2*u(18)*u(9)*u(13)*u(4)*u(17)*u(8)+u(18)*u(9)*u(13)*u(4)*u(16)*u(7)-u(18)*u(9)*u(12)*u(2)*u(14)*u(6)-u(18)*u(9)^2*u(12)*u(2)*u(17)-u(18)*u(9)*u(15)*u(5)*u(11)*u(3)-u(18)*u(9)^2*u(15)*u(5)*u(17)-u(18)^2*u(9)*u(8)*u(11)*u(3)-u(18)^2*u(9)*u(8)*u(14)*u(6)+2*u(17)*u(8)*u(10)*u(1)*u(13)*u(4)+u(17)*u(8)*u(10)*u(1)*u(16)*u(7)+u(17)*u(8)*u(13)*u(4)*u(16)*u(7)+u(17)*u(8)*u(18)*u(9)*u(11)*u(2)+u(17)*u(8)*u(18)*u(9)*u(14)*u(5)-u(17)*u(8)*u(12)*u(2)*u(14)*u(6)-u(17)^2*u(8)*u(12)*u(2)*u(9)-u(17)*u(8)*u(15)*u(5)*u(11)*u(3)-u(17)^2*u(8)*u(15)*u(5)*u(9)-u(17)*u(8)^2*u(18)*u(11)*u(3)-u(17)*u(8)^2*u(18)*u(14)*u(6)-u(10)^2*u(2)*u(14)*u(4)*u(1)-u(10)*u(2)*u(14)*u(4)*u(17)*u(8)-u(10)*u(2)*u(14)*u(4)*u(16)*u(7)-u(10)*u(2)^2*u(17)*u(7)*u(11)-u(10)^2*u(2)*u(17)*u(7)*u(1)-u(10)*u(2)*u(17)*u(7)*u(14)*u(5)-u(10)*u(2)*u(17)*u(7)*u(13)*u(4)-u(10)*u(2)*u(12)*u(1)*u(14)*u(6)-u(10)*u(2)*u(12)*u(1)*u(17)*u(9)-u(10)*u(2)*u(15)*u(4)*u(11)*u(3)-u(10)*u(2)*u(15)*u(4)*u(14)*u(6)-u(10)*u(2)*u(15)*u(4)*u(17)*u(9)-u(10)*u(2)*u(18)*u(7)*u(11)*u(3)-u(10)*u(2)*u(18)*u(7)*u(14)*u(6)-u(10)*u(2)*u(18)*u(7)*u(17)*u(9)-u(13)*u(5)*u(11)^2*u(1)*u(2)-u(13)*u(5)*u(11)*u(1)^2*u(10)-u(13)*u(5)*u(17)*u(7)^2*u(16)-u(13)*u(5)*u(17)^2*u(7)*u(8)-u(13)*u(5)^2*u(11)*u(1)*u(14)-u(13)^2*u(5)*u(11)*u(1)*u(4)-u(13)*u(5)*u(11)*u(1)*u(17)*u(8)-u(13)*u(5)*u(11)*u(1)*u(16)*u(7)-u(13)*u(5)*u(17)*u(7)*u(11)*u(2)-u(13)*u(5)*u(17)*u(7)*u(10)*u(1)-u(13)*u(5)^2*u(17)*u(7)*u(14)-u(13)^2*u(5)*u(17)*u(7)*u(4)-u(13)*u(5)*u(12)*u(1)*u(11)*u(3)-u(13)*u(5)*u(12)*u(1)*u(14)*u(6)-u(13)*u(5)*u(12)*u(1)*u(17)*u(9)-u(13)*u(5)*u(15)*u(4)*u(11)*u(3)-u(13)*u(5)*u(15)*u(4)*u(17)*u(9)-u(13)*u(5)*u(18)*u(7)*u(11)*u(3)-u(13)*u(5)*u(18)*u(7)*u(14)*u(6)-u(13)*u(5)*u(18)*u(7)*u(17)*u(9)-u(16)*u(8)*u(14)^2*u(4)*u(5)-u(16)*u(8)*u(11)^2*u(1)*u(2)-u(16)*u(8)*u(14)*u(4)^2*u(13)-u(16)*u(8)*u(11)*u(1)^2*u(10)-u(16)*u(8)*u(11)*u(1)*u(14)*u(5)-u(16)*u(8)*u(11)*u(1)*u(13)*u(4)-u(16)*u(8)^2*u(11)*u(1)*u(17)-u(16)^2*u(8)*u(11)*u(1)*u(7)-u(16)*u(8)*u(14)*u(4)*u(11)*u(2)-u(16)*u(8)*u(14)*u(4)*u(10)*u(1)-u(16)*u(8)^2*u(14)*u(4)*u(17)-u(16)^2*u(8)*u(14)*u(4)*u(7)-u(16)*u(8)*u(12)*u(1)*u(11)*u(3)-u(16)*u(8)*u(12)*u(1)*u(14)*u(6)-u(16)*u(8)*u(12)*u(1)*u(17)*u(9)-u(16)*u(8)*u(15)*u(4)*u(11)*u(3)-u(16)*u(8)*u(15)*u(4)*u(14)*u(6)-u(16)*u(8)*u(15)*u(4)*u(17)*u(9)-u(16)*u(8)*u(18)*u(7)*u(11)*u(3)-u(16)*u(8)*u(18)*u(7)*u(14)*u(6)-u(10)*u(3)*u(15)^2*u(4)*u(6)-u(10)*u(3)*u(15)*u(4)^2*u(13)-u(10)*u(3)*u(18)^2*u(7)*u(9)-u(10)*u(3)*u(18)*u(7)^2*u(16)-u(10)*u(3)*u(11)*u(1)*u(15)*u(5)-u(10)*u(3)*u(11)*u(1)*u(18)*u(8)-u(10)*u(3)*u(14)*u(4)*u(12)*u(2)-u(10)*u(3)*u(14)*u(4)*u(15)*u(5)-u(10)*u(3)*u(14)*u(4)*u(18)*u(8)-u(10)*u(3)*u(17)*u(7)*u(12)*u(2)-u(10)*u(3)*u(17)*u(7)*u(15)*u(5)-u(10)*u(3)*u(17)*u(7)*u(18)*u(8)-u(10)*u(3)^2*u(15)*u(4)*u(12)-u(10)^2*u(3)*u(15)*u(4)*u(1)-u(10)*u(3)*u(15)*u(4)*u(18)*u(9)-u(10)*u(3)*u(15)*u(4)*u(16)*u(7)-u(10)*u(3)^2*u(18)*u(7)*u(12)-u(10)^2*u(3)*u(18)*u(7)*u(1)-u(10)*u(3)*u(18)*u(7)*u(15)*u(6)-u(10)*u(3)*u(18)*u(7)*u(13)*u(4)-u(13)*u(6)*u(12)*u(1)^2*u(10)-u(13)*u(6)*u(12)^2*u(1)*u(3)-u(13)*u(6)*u(18)^2*u(7)*u(9)-u(13)*u(6)*u(18)*u(7)^2*u(16)-u(13)*u(6)*u(11)*u(1)*u(12)*u(2)-u(13)*u(6)*u(11)*u(1)*u(15)*u(5)-u(13)*u(6)*u(11)*u(1)*u(18)*u(8)-u(13)*u(6)*u(14)*u(4)*u(12)*u(2)-u(13)*u(6)*u(14)*u(4)*u(18)*u(8)-u(13)*u(6)*u(17)*u(7)*u(12)*u(2)-u(13)*u(6)*u(17)*u(7)*u(15)*u(5)-u(13)*u(6)*u(17)*u(7)*u(18)*u(8)-u(13)*u(6)^2*u(12)*u(1)*u(15)-u(13)^2*u(6)*u(12)*u(1)*u(4)-u(13)*u(6)*u(12)*u(1)*u(18)*u(9)-u(13)*u(6)*u(12)*u(1)*u(16)*u(7)-u(13)*u(6)*u(18)*u(7)*u(12)*u(3)-u(13)*u(6)*u(18)*u(7)*u(10)*u(1)-u(13)*u(6)^2*u(18)*u(7)*u(15)-u(13)^2*u(6)*u(18)*u(7)*u(4)-u(16)*u(9)*u(12)*u(1)^2*u(10)-u(16)*u(9)*u(12)^2*u(1)*u(3)-u(16)*u(9)*u(15)^2*u(4)*u(6)-u(16)*u(9)*u(15)*u(4)^2*u(13)-u(16)*u(9)*u(11)*u(1)*u(12)*u(2)-u(16)*u(9)*u(11)*u(1)*u(15)*u(5)-u(16)*u(9)*u(11)*u(1)*u(18)*u(8)-u(16)*u(9)*u(14)*u(4)*u(12)*u(2)-u(16)*u(9)*u(14)*u(4)*u(15)*u(5)-u(16)*u(9)*u(14)*u(4)*u(18)*u(8)-u(16)*u(9)*u(17)*u(7)*u(12)*u(2)-u(16)*u(9)*u(17)*u(7)*u(15)*u(5)-u(16)*u(9)*u(12)*u(1)*u(15)*u(6)-u(16)*u(9)*u(12)*u(1)*u(13)*u(4)-u(16)*u(9)^2*u(12)*u(1)*u(18)-u(16)^2*u(9)*u(12)*u(1)*u(7)-u(16)*u(9)*u(15)*u(4)*u(12)*u(3)-u(16)*u(9)*u(15)*u(4)*u(10)*u(1)-u(16)*u(9)^2*u(15)*u(4)*u(18)-u(16)^2*u(9)*u(15)*u(4)*u(7))*u(20)+2*(u(12)^2*u(3)*u(2)+u(18)^2*u(9)*u(8)+u(17)*u(8)^2*u(18)+u(11)*u(2)^2*u(12)+u(14)*u(5)^2*u(15)+u(15)^2*u(6)*u(5)+u(12)*u(3)*u(15)*u(5)+u(12)*u(3)*u(18)*u(8)+u(11)*u(2)*u(15)*u(5)+u(11)*u(2)*u(18)*u(8)+u(15)*u(6)*u(12)*u(2)+u(15)*u(6)*u(18)*u(8)+u(14)*u(5)*u(12)*u(2)+u(14)*u(5)*u(18)*u(8)+u(18)*u(9)*u(12)*u(2)+u(18)*u(9)*u(15)*u(5)+u(17)*u(8)*u(12)*u(2)+u(17)*u(8)*u(15)*u(5)+u(12)*u(1)*u(10)*u(2)+u(12)*u(1)*u(13)*u(5)+u(12)*u(1)*u(16)*u(8)+u(15)*u(4)*u(10)*u(2)+u(15)*u(4)*u(13)*u(5)+u(15)*u(4)*u(16)*u(8)+u(18)*u(7)*u(10)*u(2)+u(18)*u(7)*u(13)*u(5)+u(18)*u(7)*u(16)*u(8))/(u(12)*u(3)*u(13)^2*u(4)^2+u(12)*u(3)*u(16)^2*u(7)^2+u(12)^2*u(3)^2*u(14)*u(5)+u(12)^2*u(3)^2*u(13)*u(4)+u(12)^2*u(3)^2*u(17)*u(8)+u(12)^2*u(3)^2*u(16)*u(7)+u(11)*u(2)*u(13)^2*u(4)^2+u(11)*u(2)*u(16)^2*u(7)^2+u(11)^2*u(2)^2*u(15)*u(6)+u(11)^2*u(2)^2*u(13)*u(4)+u(11)^2*u(2)^2*u(18)*u(9)+u(11)^2*u(2)^2*u(16)*u(7)+u(15)*u(6)*u(10)^2*u(1)^2+u(15)*u(6)*u(16)^2*u(7)^2+u(15)^2*u(6)^2*u(11)*u(2)+u(15)^2*u(6)^2*u(10)*u(1)+u(15)^2*u(6)^2*u(17)*u(8)+u(15)^2*u(6)^2*u(16)*u(7)+u(14)*u(5)*u(10)^2*u(1)^2+u(14)*u(5)*u(16)^2*u(7)^2+u(14)^2*u(5)^2*u(12)*u(3)+u(14)^2*u(5)^2*u(10)*u(1)+u(14)^2*u(5)^2*u(18)*u(9)+u(14)^2*u(5)^2*u(16)*u(7)+u(18)*u(9)*u(10)^2*u(1)^2+u(18)*u(9)*u(13)^2*u(4)^2+u(18)^2*u(9)^2*u(11)*u(2)+u(18)^2*u(9)^2*u(10)*u(1)+u(18)^2*u(9)^2*u(14)*u(5)+u(18)^2*u(9)^2*u(13)*u(4)+u(17)*u(8)*u(10)^2*u(1)^2+u(17)*u(8)*u(13)^2*u(4)^2+u(17)^2*u(8)^2*u(12)*u(3)+u(17)^2*u(8)^2*u(10)*u(1)+u(17)^2*u(8)^2*u(15)*u(6)+u(17)^2*u(8)^2*u(13)*u(4)-u(10)*u(2)*u(14)^2*u(4)*u(5)-u(10)*u(2)*u(14)*u(4)^2*u(13)-u(10)*u(2)*u(17)*u(7)^2*u(16)-u(10)*u(2)*u(17)^2*u(7)*u(8)-u(10)*u(2)^2*u(14)*u(4)*u(11)+2*u(12)*u(3)*u(10)*u(1)*u(14)*u(5)+u(12)*u(3)*u(10)*u(1)*u(13)*u(4)+2*u(12)*u(3)*u(10)*u(1)*u(17)*u(8)+u(12)*u(3)*u(10)*u(1)*u(16)*u(7)+u(12)*u(3)*u(15)*u(6)*u(11)*u(2)+u(12)*u(3)*u(15)*u(6)*u(10)*u(1)+u(12)*u(3)*u(15)*u(6)*u(13)*u(4)+2*u(12)*u(3)*u(15)*u(6)*u(17)*u(8)+2*u(12)*u(3)*u(15)*u(6)*u(16)*u(7)+2*u(12)*u(3)*u(13)*u(4)*u(11)*u(2)+2*u(12)*u(3)*u(13)*u(4)*u(14)*u(5)+2*u(12)*u(3)*u(13)*u(4)*u(17)*u(8)+2*u(12)*u(3)*u(13)*u(4)*u(16)*u(7)+u(12)*u(3)*u(18)*u(9)*u(11)*u(2)+u(12)*u(3)*u(18)*u(9)*u(10)*u(1)+2*u(12)*u(3)*u(18)*u(9)*u(14)*u(5)+2*u(12)*u(3)*u(18)*u(9)*u(13)*u(4)+u(12)*u(3)*u(18)*u(9)*u(16)*u(7)+2*u(12)*u(3)*u(16)*u(7)*u(11)*u(2)+2*u(12)*u(3)*u(16)*u(7)*u(14)*u(5)+2*u(12)*u(3)*u(16)*u(7)*u(17)*u(8)-u(12)^2*u(3)*u(2)*u(14)*u(6)-u(12)^2*u(3)*u(2)*u(17)*u(9)-u(12)*u(3)^2*u(15)*u(5)*u(11)-u(12)*u(3)*u(15)*u(5)*u(17)*u(9)-u(12)*u(3)^2*u(18)*u(8)*u(11)-u(12)*u(3)*u(18)*u(8)*u(14)*u(6)+u(11)*u(2)*u(12)*u(3)*u(14)*u(5)+u(11)*u(2)*u(12)*u(3)*u(17)*u(8)+u(11)*u(2)*u(10)*u(1)*u(14)*u(5)+u(11)*u(2)*u(10)*u(1)*u(13)*u(4)+u(11)*u(2)*u(10)*u(1)*u(17)*u(8)+u(11)*u(2)*u(10)*u(1)*u(16)*u(7)+2*u(11)*u(2)*u(15)*u(6)*u(10)*u(1)+2*u(11)*u(2)*u(15)*u(6)*u(13)*u(4)+2*u(11)*u(2)*u(15)*u(6)*u(17)*u(8)+2*u(11)*u(2)*u(15)*u(6)*u(16)*u(7)+u(11)*u(2)*u(13)*u(4)*u(14)*u(5)+2*u(11)*u(2)*u(13)*u(4)*u(17)*u(8)+2*u(11)*u(2)*u(13)*u(4)*u(16)*u(7)+2*u(11)*u(2)*u(18)*u(9)*u(10)*u(1)+2*u(11)*u(2)*u(18)*u(9)*u(14)*u(5)+2*u(11)*u(2)*u(18)*u(9)*u(13)*u(4)+2*u(11)*u(2)*u(18)*u(9)*u(16)*u(7)+2*u(11)*u(2)*u(16)*u(7)*u(14)*u(5)+u(11)*u(2)*u(16)*u(7)*u(17)*u(8)-u(11)*u(2)^2*u(12)*u(14)*u(6)-u(11)*u(2)^2*u(12)*u(17)*u(9)-u(11)^2*u(2)*u(15)*u(5)*u(3)-u(11)*u(2)*u(15)*u(5)*u(17)*u(9)-u(11)^2*u(2)*u(18)*u(8)*u(3)-u(11)*u(2)*u(18)*u(8)*u(14)*u(6)+u(15)*u(6)*u(12)*u(3)*u(14)*u(5)+2*u(15)*u(6)*u(10)*u(1)*u(14)*u(5)+u(15)*u(6)*u(10)*u(1)*u(13)*u(4)+2*u(15)*u(6)*u(10)*u(1)*u(17)*u(8)+2*u(15)*u(6)*u(10)*u(1)*u(16)*u(7)+2*u(15)*u(6)*u(13)*u(4)*u(17)*u(8)+u(15)*u(6)*u(13)*u(4)*u(16)*u(7)+2*u(15)*u(6)*u(18)*u(9)*u(11)*u(2)+2*u(15)*u(6)*u(18)*u(9)*u(10)*u(1)+u(15)*u(6)*u(18)*u(9)*u(14)*u(5)+u(15)*u(6)*u(18)*u(9)*u(13)*u(4)+u(15)*u(6)*u(18)*u(9)*u(16)*u(7)+2*u(15)*u(6)*u(16)*u(7)*u(14)*u(5)+2*u(15)*u(6)*u(16)*u(7)*u(17)*u(8)-u(15)*u(6)^2*u(12)*u(2)*u(14)-u(15)*u(6)*u(12)*u(2)*u(17)*u(9)-u(15)^2*u(6)*u(5)*u(11)*u(3)-u(15)^2*u(6)*u(5)*u(17)*u(9)-u(15)*u(6)*u(18)*u(8)*u(11)*u(3)-u(15)*u(6)^2*u(18)*u(8)*u(14)+2*u(14)*u(5)*u(12)*u(3)*u(17)*u(8)+u(14)*u(5)*u(10)*u(1)*u(13)*u(4)+2*u(14)*u(5)*u(10)*u(1)*u(17)*u(8)+2*u(14)*u(5)*u(10)*u(1)*u(16)*u(7)+u(14)*u(5)*u(15)*u(6)*u(11)*u(2)+u(14)*u(5)*u(15)*u(6)*u(17)*u(8)+u(14)*u(5)*u(13)*u(4)*u(17)*u(8)+u(14)*u(5)*u(13)*u(4)*u(16)*u(7)+2*u(14)*u(5)*u(18)*u(9)*u(10)*u(1)+2*u(14)*u(5)*u(18)*u(9)*u(13)*u(4)+2*u(14)*u(5)*u(18)*u(9)*u(16)*u(7)+u(14)*u(5)*u(16)*u(7)*u(17)*u(8)-u(14)^2*u(5)*u(12)*u(2)*u(6)-u(14)*u(5)*u(12)*u(2)*u(17)*u(9)-u(14)*u(5)^2*u(15)*u(11)*u(3)-u(14)*u(5)^2*u(15)*u(17)*u(9)-u(14)*u(5)*u(18)*u(8)*u(11)*u(3)-u(14)^2*u(5)*u(18)*u(8)*u(6)+u(18)*u(9)*u(12)*u(3)*u(17)*u(8)+2*u(18)*u(9)*u(10)*u(1)*u(13)*u(4)+2*u(18)*u(9)*u(10)*u(1)*u(17)*u(8)+u(18)*u(9)*u(10)*u(1)*u(16)*u(7)+u(18)*u(9)*u(15)*u(6)*u(17)*u(8)+2*u(18)*u(9)*u(13)*u(4)*u(17)*u(8)+u(18)*u(9)*u(13)*u(4)*u(16)*u(7)-u(18)*u(9)*u(12)*u(2)*u(14)*u(6)-u(18)*u(9)^2*u(12)*u(2)*u(17)-u(18)*u(9)*u(15)*u(5)*u(11)*u(3)-u(18)*u(9)^2*u(15)*u(5)*u(17)-u(18)^2*u(9)*u(8)*u(11)*u(3)-u(18)^2*u(9)*u(8)*u(14)*u(6)+2*u(17)*u(8)*u(10)*u(1)*u(13)*u(4)+u(17)*u(8)*u(10)*u(1)*u(16)*u(7)+u(17)*u(8)*u(13)*u(4)*u(16)*u(7)+u(17)*u(8)*u(18)*u(9)*u(11)*u(2)+u(17)*u(8)*u(18)*u(9)*u(14)*u(5)-u(17)*u(8)*u(12)*u(2)*u(14)*u(6)-u(17)^2*u(8)*u(12)*u(2)*u(9)-u(17)*u(8)*u(15)*u(5)*u(11)*u(3)-u(17)^2*u(8)*u(15)*u(5)*u(9)-u(17)*u(8)^2*u(18)*u(11)*u(3)-u(17)*u(8)^2*u(18)*u(14)*u(6)-u(10)^2*u(2)*u(14)*u(4)*u(1)-u(10)*u(2)*u(14)*u(4)*u(17)*u(8)-u(10)*u(2)*u(14)*u(4)*u(16)*u(7)-u(10)*u(2)^2*u(17)*u(7)*u(11)-u(10)^2*u(2)*u(17)*u(7)*u(1)-u(10)*u(2)*u(17)*u(7)*u(14)*u(5)-u(10)*u(2)*u(17)*u(7)*u(13)*u(4)-u(10)*u(2)*u(12)*u(1)*u(14)*u(6)-u(10)*u(2)*u(12)*u(1)*u(17)*u(9)-u(10)*u(2)*u(15)*u(4)*u(11)*u(3)-u(10)*u(2)*u(15)*u(4)*u(14)*u(6)-u(10)*u(2)*u(15)*u(4)*u(17)*u(9)-u(10)*u(2)*u(18)*u(7)*u(11)*u(3)-u(10)*u(2)*u(18)*u(7)*u(14)*u(6)-u(10)*u(2)*u(18)*u(7)*u(17)*u(9)-u(13)*u(5)*u(11)^2*u(1)*u(2)-u(13)*u(5)*u(11)*u(1)^2*u(10)-u(13)*u(5)*u(17)*u(7)^2*u(16)-u(13)*u(5)*u(17)^2*u(7)*u(8)-u(13)*u(5)^2*u(11)*u(1)*u(14)-u(13)^2*u(5)*u(11)*u(1)*u(4)-u(13)*u(5)*u(11)*u(1)*u(17)*u(8)-u(13)*u(5)*u(11)*u(1)*u(16)*u(7)-u(13)*u(5)*u(17)*u(7)*u(11)*u(2)-u(13)*u(5)*u(17)*u(7)*u(10)*u(1)-u(13)*u(5)^2*u(17)*u(7)*u(14)-u(13)^2*u(5)*u(17)*u(7)*u(4)-u(13)*u(5)*u(12)*u(1)*u(11)*u(3)-u(13)*u(5)*u(12)*u(1)*u(14)*u(6)-u(13)*u(5)*u(12)*u(1)*u(17)*u(9)-u(13)*u(5)*u(15)*u(4)*u(11)*u(3)-u(13)*u(5)*u(15)*u(4)*u(17)*u(9)-u(13)*u(5)*u(18)*u(7)*u(11)*u(3)-u(13)*u(5)*u(18)*u(7)*u(14)*u(6)-u(13)*u(5)*u(18)*u(7)*u(17)*u(9)-u(16)*u(8)*u(14)^2*u(4)*u(5)-u(16)*u(8)*u(11)^2*u(1)*u(2)-u(16)*u(8)*u(14)*u(4)^2*u(13)-u(16)*u(8)*u(11)*u(1)^2*u(10)-u(16)*u(8)*u(11)*u(1)*u(14)*u(5)-u(16)*u(8)*u(11)*u(1)*u(13)*u(4)-u(16)*u(8)^2*u(11)*u(1)*u(17)-u(16)^2*u(8)*u(11)*u(1)*u(7)-u(16)*u(8)*u(14)*u(4)*u(11)*u(2)-u(16)*u(8)*u(14)*u(4)*u(10)*u(1)-u(16)*u(8)^2*u(14)*u(4)*u(17)-u(16)^2*u(8)*u(14)*u(4)*u(7)-u(16)*u(8)*u(12)*u(1)*u(11)*u(3)-u(16)*u(8)*u(12)*u(1)*u(14)*u(6)-u(16)*u(8)*u(12)*u(1)*u(17)*u(9)-u(16)*u(8)*u(15)*u(4)*u(11)*u(3)-u(16)*u(8)*u(15)*u(4)*u(14)*u(6)-u(16)*u(8)*u(15)*u(4)*u(17)*u(9)-u(16)*u(8)*u(18)*u(7)*u(11)*u(3)-u(16)*u(8)*u(18)*u(7)*u(14)*u(6)-u(10)*u(3)*u(15)^2*u(4)*u(6)-u(10)*u(3)*u(15)*u(4)^2*u(13)-u(10)*u(3)*u(18)^2*u(7)*u(9)-u(10)*u(3)*u(18)*u(7)^2*u(16)-u(10)*u(3)*u(11)*u(1)*u(15)*u(5)-u(10)*u(3)*u(11)*u(1)*u(18)*u(8)-u(10)*u(3)*u(14)*u(4)*u(12)*u(2)-u(10)*u(3)*u(14)*u(4)*u(15)*u(5)-u(10)*u(3)*u(14)*u(4)*u(18)*u(8)-u(10)*u(3)*u(17)*u(7)*u(12)*u(2)-u(10)*u(3)*u(17)*u(7)*u(15)*u(5)-u(10)*u(3)*u(17)*u(7)*u(18)*u(8)-u(10)*u(3)^2*u(15)*u(4)*u(12)-u(10)^2*u(3)*u(15)*u(4)*u(1)-u(10)*u(3)*u(15)*u(4)*u(18)*u(9)-u(10)*u(3)*u(15)*u(4)*u(16)*u(7)-u(10)*u(3)^2*u(18)*u(7)*u(12)-u(10)^2*u(3)*u(18)*u(7)*u(1)-u(10)*u(3)*u(18)*u(7)*u(15)*u(6)-u(10)*u(3)*u(18)*u(7)*u(13)*u(4)-u(13)*u(6)*u(12)*u(1)^2*u(10)-u(13)*u(6)*u(12)^2*u(1)*u(3)-u(13)*u(6)*u(18)^2*u(7)*u(9)-u(13)*u(6)*u(18)*u(7)^2*u(16)-u(13)*u(6)*u(11)*u(1)*u(12)*u(2)-u(13)*u(6)*u(11)*u(1)*u(15)*u(5)-u(13)*u(6)*u(11)*u(1)*u(18)*u(8)-u(13)*u(6)*u(14)*u(4)*u(12)*u(2)-u(13)*u(6)*u(14)*u(4)*u(18)*u(8)-u(13)*u(6)*u(17)*u(7)*u(12)*u(2)-u(13)*u(6)*u(17)*u(7)*u(15)*u(5)-u(13)*u(6)*u(17)*u(7)*u(18)*u(8)-u(13)*u(6)^2*u(12)*u(1)*u(15)-u(13)^2*u(6)*u(12)*u(1)*u(4)-u(13)*u(6)*u(12)*u(1)*u(18)*u(9)-u(13)*u(6)*u(12)*u(1)*u(16)*u(7)-u(13)*u(6)*u(18)*u(7)*u(12)*u(3)-u(13)*u(6)*u(18)*u(7)*u(10)*u(1)-u(13)*u(6)^2*u(18)*u(7)*u(15)-u(13)^2*u(6)*u(18)*u(7)*u(4)-u(16)*u(9)*u(12)*u(1)^2*u(10)-u(16)*u(9)*u(12)^2*u(1)*u(3)-u(16)*u(9)*u(15)^2*u(4)*u(6)-u(16)*u(9)*u(15)*u(4)^2*u(13)-u(16)*u(9)*u(11)*u(1)*u(12)*u(2)-u(16)*u(9)*u(11)*u(1)*u(15)*u(5)-u(16)*u(9)*u(11)*u(1)*u(18)*u(8)-u(16)*u(9)*u(14)*u(4)*u(12)*u(2)-u(16)*u(9)*u(14)*u(4)*u(15)*u(5)-u(16)*u(9)*u(14)*u(4)*u(18)*u(8)-u(16)*u(9)*u(17)*u(7)*u(12)*u(2)-u(16)*u(9)*u(17)*u(7)*u(15)*u(5)-u(16)*u(9)*u(12)*u(1)*u(15)*u(6)-u(16)*u(9)*u(12)*u(1)*u(13)*u(4)-u(16)*u(9)^2*u(12)*u(1)*u(18)-u(16)^2*u(9)*u(12)*u(1)*u(7)-u(16)*u(9)*u(15)*u(4)*u(12)*u(3)-u(16)*u(9)*u(15)*u(4)*u(10)*u(1)-u(16)*u(9)^2*u(15)*u(4)*u(18)-u(16)^2*u(9)*u(15)*u(4)*u(7))*u(21)
  invL3 : Fcn  Expr=2*(u(16)^2*u(7)*u(9)+u(13)^2*u(4)*u(6)+u(10)^2*u(1)*u(3)+u(15)*u(6)^2*u(13)+u(18)*u(9)^2*u(16)+u(12)*u(3)^2*u(10)+u(10)*u(2)*u(11)*u(3)+u(10)*u(2)*u(14)*u(6)+u(10)*u(2)*u(17)*u(9)+u(13)*u(5)*u(11)*u(3)+u(13)*u(5)*u(14)*u(6)+u(13)*u(5)*u(17)*u(9)+u(16)*u(8)*u(11)*u(3)+u(16)*u(8)*u(14)*u(6)+u(16)*u(8)*u(17)*u(9)+u(12)*u(3)*u(13)*u(6)+u(12)*u(3)*u(16)*u(9)+u(10)*u(1)*u(13)*u(6)+u(10)*u(1)*u(16)*u(9)+u(15)*u(6)*u(10)*u(3)+u(15)*u(6)*u(16)*u(9)+u(13)*u(4)*u(10)*u(3)+u(13)*u(4)*u(16)*u(9)+u(18)*u(9)*u(10)*u(3)+u(18)*u(9)*u(13)*u(6)+u(16)*u(7)*u(10)*u(3)+u(16)*u(7)*u(13)*u(6))/(u(12)*u(3)*u(13)^2*u(4)^2+u(12)*u(3)*u(16)^2*u(7)^2+u(12)^2*u(3)^2*u(14)*u(5)+u(12)^2*u(3)^2*u(13)*u(4)+u(12)^2*u(3)^2*u(17)*u(8)+u(12)^2*u(3)^2*u(16)*u(7)+u(11)*u(2)*u(13)^2*u(4)^2+u(11)*u(2)*u(16)^2*u(7)^2+u(11)^2*u(2)^2*u(15)*u(6)+u(11)^2*u(2)^2*u(13)*u(4)+u(11)^2*u(2)^2*u(18)*u(9)+u(11)^2*u(2)^2*u(16)*u(7)+u(15)*u(6)*u(10)^2*u(1)^2+u(15)*u(6)*u(16)^2*u(7)^2+u(15)^2*u(6)^2*u(11)*u(2)+u(15)^2*u(6)^2*u(10)*u(1)+u(15)^2*u(6)^2*u(17)*u(8)+u(15)^2*u(6)^2*u(16)*u(7)+u(14)*u(5)*u(10)^2*u(1)^2+u(14)*u(5)*u(16)^2*u(7)^2+u(14)^2*u(5)^2*u(12)*u(3)+u(14)^2*u(5)^2*u(10)*u(1)+u(14)^2*u(5)^2*u(18)*u(9)+u(14)^2*u(5)^2*u(16)*u(7)+u(18)*u(9)*u(10)^2*u(1)^2+u(18)*u(9)*u(13)^2*u(4)^2+u(18)^2*u(9)^2*u(11)*u(2)+u(18)^2*u(9)^2*u(10)*u(1)+u(18)^2*u(9)^2*u(14)*u(5)+u(18)^2*u(9)^2*u(13)*u(4)+u(17)*u(8)*u(10)^2*u(1)^2+u(17)*u(8)*u(13)^2*u(4)^2+u(17)^2*u(8)^2*u(12)*u(3)+u(17)^2*u(8)^2*u(10)*u(1)+u(17)^2*u(8)^2*u(15)*u(6)+u(17)^2*u(8)^2*u(13)*u(4)-u(10)*u(2)*u(14)^2*u(4)*u(5)-u(10)*u(2)*u(14)*u(4)^2*u(13)-u(10)*u(2)*u(17)*u(7)^2*u(16)-u(10)*u(2)*u(17)^2*u(7)*u(8)-u(10)*u(2)^2*u(14)*u(4)*u(11)+2*u(12)*u(3)*u(10)*u(1)*u(14)*u(5)+u(12)*u(3)*u(10)*u(1)*u(13)*u(4)+2*u(12)*u(3)*u(10)*u(1)*u(17)*u(8)+u(12)*u(3)*u(10)*u(1)*u(16)*u(7)+u(12)*u(3)*u(15)*u(6)*u(11)*u(2)+u(12)*u(3)*u(15)*u(6)*u(10)*u(1)+u(12)*u(3)*u(15)*u(6)*u(13)*u(4)+2*u(12)*u(3)*u(15)*u(6)*u(17)*u(8)+2*u(12)*u(3)*u(15)*u(6)*u(16)*u(7)+2*u(12)*u(3)*u(13)*u(4)*u(11)*u(2)+2*u(12)*u(3)*u(13)*u(4)*u(14)*u(5)+2*u(12)*u(3)*u(13)*u(4)*u(17)*u(8)+2*u(12)*u(3)*u(13)*u(4)*u(16)*u(7)+u(12)*u(3)*u(18)*u(9)*u(11)*u(2)+u(12)*u(3)*u(18)*u(9)*u(10)*u(1)+2*u(12)*u(3)*u(18)*u(9)*u(14)*u(5)+2*u(12)*u(3)*u(18)*u(9)*u(13)*u(4)+u(12)*u(3)*u(18)*u(9)*u(16)*u(7)+2*u(12)*u(3)*u(16)*u(7)*u(11)*u(2)+2*u(12)*u(3)*u(16)*u(7)*u(14)*u(5)+2*u(12)*u(3)*u(16)*u(7)*u(17)*u(8)-u(12)^2*u(3)*u(2)*u(14)*u(6)-u(12)^2*u(3)*u(2)*u(17)*u(9)-u(12)*u(3)^2*u(15)*u(5)*u(11)-u(12)*u(3)*u(15)*u(5)*u(17)*u(9)-u(12)*u(3)^2*u(18)*u(8)*u(11)-u(12)*u(3)*u(18)*u(8)*u(14)*u(6)+u(11)*u(2)*u(12)*u(3)*u(14)*u(5)+u(11)*u(2)*u(12)*u(3)*u(17)*u(8)+u(11)*u(2)*u(10)*u(1)*u(14)*u(5)+u(11)*u(2)*u(10)*u(1)*u(13)*u(4)+u(11)*u(2)*u(10)*u(1)*u(17)*u(8)+u(11)*u(2)*u(10)*u(1)*u(16)*u(7)+2*u(11)*u(2)*u(15)*u(6)*u(10)*u(1)+2*u(11)*u(2)*u(15)*u(6)*u(13)*u(4)+2*u(11)*u(2)*u(15)*u(6)*u(17)*u(8)+2*u(11)*u(2)*u(15)*u(6)*u(16)*u(7)+u(11)*u(2)*u(13)*u(4)*u(14)*u(5)+2*u(11)*u(2)*u(13)*u(4)*u(17)*u(8)+2*u(11)*u(2)*u(13)*u(4)*u(16)*u(7)+2*u(11)*u(2)*u(18)*u(9)*u(10)*u(1)+2*u(11)*u(2)*u(18)*u(9)*u(14)*u(5)+2*u(11)*u(2)*u(18)*u(9)*u(13)*u(4)+2*u(11)*u(2)*u(18)*u(9)*u(16)*u(7)+2*u(11)*u(2)*u(16)*u(7)*u(14)*u(5)+u(11)*u(2)*u(16)*u(7)*u(17)*u(8)-u(11)*u(2)^2*u(12)*u(14)*u(6)-u(11)*u(2)^2*u(12)*u(17)*u(9)-u(11)^2*u(2)*u(15)*u(5)*u(3)-u(11)*u(2)*u(15)*u(5)*u(17)*u(9)-u(11)^2*u(2)*u(18)*u(8)*u(3)-u(11)*u(2)*u(18)*u(8)*u(14)*u(6)+u(15)*u(6)*u(12)*u(3)*u(14)*u(5)+2*u(15)*u(6)*u(10)*u(1)*u(14)*u(5)+u(15)*u(6)*u(10)*u(1)*u(13)*u(4)+2*u(15)*u(6)*u(10)*u(1)*u(17)*u(8)+2*u(15)*u(6)*u(10)*u(1)*u(16)*u(7)+2*u(15)*u(6)*u(13)*u(4)*u(17)*u(8)+u(15)*u(6)*u(13)*u(4)*u(16)*u(7)+2*u(15)*u(6)*u(18)*u(9)*u(11)*u(2)+2*u(15)*u(6)*u(18)*u(9)*u(10)*u(1)+u(15)*u(6)*u(18)*u(9)*u(14)*u(5)+u(15)*u(6)*u(18)*u(9)*u(13)*u(4)+u(15)*u(6)*u(18)*u(9)*u(16)*u(7)+2*u(15)*u(6)*u(16)*u(7)*u(14)*u(5)+2*u(15)*u(6)*u(16)*u(7)*u(17)*u(8)-u(15)*u(6)^2*u(12)*u(2)*u(14)-u(15)*u(6)*u(12)*u(2)*u(17)*u(9)-u(15)^2*u(6)*u(5)*u(11)*u(3)-u(15)^2*u(6)*u(5)*u(17)*u(9)-u(15)*u(6)*u(18)*u(8)*u(11)*u(3)-u(15)*u(6)^2*u(18)*u(8)*u(14)+2*u(14)*u(5)*u(12)*u(3)*u(17)*u(8)+u(14)*u(5)*u(10)*u(1)*u(13)*u(4)+2*u(14)*u(5)*u(10)*u(1)*u(17)*u(8)+2*u(14)*u(5)*u(10)*u(1)*u(16)*u(7)+u(14)*u(5)*u(15)*u(6)*u(11)*u(2)+u(14)*u(5)*u(15)*u(6)*u(17)*u(8)+u(14)*u(5)*u(13)*u(4)*u(17)*u(8)+u(14)*u(5)*u(13)*u(4)*u(16)*u(7)+2*u(14)*u(5)*u(18)*u(9)*u(10)*u(1)+2*u(14)*u(5)*u(18)*u(9)*u(13)*u(4)+2*u(14)*u(5)*u(18)*u(9)*u(16)*u(7)+u(14)*u(5)*u(16)*u(7)*u(17)*u(8)-u(14)^2*u(5)*u(12)*u(2)*u(6)-u(14)*u(5)*u(12)*u(2)*u(17)*u(9)-u(14)*u(5)^2*u(15)*u(11)*u(3)-u(14)*u(5)^2*u(15)*u(17)*u(9)-u(14)*u(5)*u(18)*u(8)*u(11)*u(3)-u(14)^2*u(5)*u(18)*u(8)*u(6)+u(18)*u(9)*u(12)*u(3)*u(17)*u(8)+2*u(18)*u(9)*u(10)*u(1)*u(13)*u(4)+2*u(18)*u(9)*u(10)*u(1)*u(17)*u(8)+u(18)*u(9)*u(10)*u(1)*u(16)*u(7)+u(18)*u(9)*u(15)*u(6)*u(17)*u(8)+2*u(18)*u(9)*u(13)*u(4)*u(17)*u(8)+u(18)*u(9)*u(13)*u(4)*u(16)*u(7)-u(18)*u(9)*u(12)*u(2)*u(14)*u(6)-u(18)*u(9)^2*u(12)*u(2)*u(17)-u(18)*u(9)*u(15)*u(5)*u(11)*u(3)-u(18)*u(9)^2*u(15)*u(5)*u(17)-u(18)^2*u(9)*u(8)*u(11)*u(3)-u(18)^2*u(9)*u(8)*u(14)*u(6)+2*u(17)*u(8)*u(10)*u(1)*u(13)*u(4)+u(17)*u(8)*u(10)*u(1)*u(16)*u(7)+u(17)*u(8)*u(13)*u(4)*u(16)*u(7)+u(17)*u(8)*u(18)*u(9)*u(11)*u(2)+u(17)*u(8)*u(18)*u(9)*u(14)*u(5)-u(17)*u(8)*u(12)*u(2)*u(14)*u(6)-u(17)^2*u(8)*u(12)*u(2)*u(9)-u(17)*u(8)*u(15)*u(5)*u(11)*u(3)-u(17)^2*u(8)*u(15)*u(5)*u(9)-u(17)*u(8)^2*u(18)*u(11)*u(3)-u(17)*u(8)^2*u(18)*u(14)*u(6)-u(10)^2*u(2)*u(14)*u(4)*u(1)-u(10)*u(2)*u(14)*u(4)*u(17)*u(8)-u(10)*u(2)*u(14)*u(4)*u(16)*u(7)-u(10)*u(2)^2*u(17)*u(7)*u(11)-u(10)^2*u(2)*u(17)*u(7)*u(1)-u(10)*u(2)*u(17)*u(7)*u(14)*u(5)-u(10)*u(2)*u(17)*u(7)*u(13)*u(4)-u(10)*u(2)*u(12)*u(1)*u(14)*u(6)-u(10)*u(2)*u(12)*u(1)*u(17)*u(9)-u(10)*u(2)*u(15)*u(4)*u(11)*u(3)-u(10)*u(2)*u(15)*u(4)*u(14)*u(6)-u(10)*u(2)*u(15)*u(4)*u(17)*u(9)-u(10)*u(2)*u(18)*u(7)*u(11)*u(3)-u(10)*u(2)*u(18)*u(7)*u(14)*u(6)-u(10)*u(2)*u(18)*u(7)*u(17)*u(9)-u(13)*u(5)*u(11)^2*u(1)*u(2)-u(13)*u(5)*u(11)*u(1)^2*u(10)-u(13)*u(5)*u(17)*u(7)^2*u(16)-u(13)*u(5)*u(17)^2*u(7)*u(8)-u(13)*u(5)^2*u(11)*u(1)*u(14)-u(13)^2*u(5)*u(11)*u(1)*u(4)-u(13)*u(5)*u(11)*u(1)*u(17)*u(8)-u(13)*u(5)*u(11)*u(1)*u(16)*u(7)-u(13)*u(5)*u(17)*u(7)*u(11)*u(2)-u(13)*u(5)*u(17)*u(7)*u(10)*u(1)-u(13)*u(5)^2*u(17)*u(7)*u(14)-u(13)^2*u(5)*u(17)*u(7)*u(4)-u(13)*u(5)*u(12)*u(1)*u(11)*u(3)-u(13)*u(5)*u(12)*u(1)*u(14)*u(6)-u(13)*u(5)*u(12)*u(1)*u(17)*u(9)-u(13)*u(5)*u(15)*u(4)*u(11)*u(3)-u(13)*u(5)*u(15)*u(4)*u(17)*u(9)-u(13)*u(5)*u(18)*u(7)*u(11)*u(3)-u(13)*u(5)*u(18)*u(7)*u(14)*u(6)-u(13)*u(5)*u(18)*u(7)*u(17)*u(9)-u(16)*u(8)*u(14)^2*u(4)*u(5)-u(16)*u(8)*u(11)^2*u(1)*u(2)-u(16)*u(8)*u(14)*u(4)^2*u(13)-u(16)*u(8)*u(11)*u(1)^2*u(10)-u(16)*u(8)*u(11)*u(1)*u(14)*u(5)-u(16)*u(8)*u(11)*u(1)*u(13)*u(4)-u(16)*u(8)^2*u(11)*u(1)*u(17)-u(16)^2*u(8)*u(11)*u(1)*u(7)-u(16)*u(8)*u(14)*u(4)*u(11)*u(2)-u(16)*u(8)*u(14)*u(4)*u(10)*u(1)-u(16)*u(8)^2*u(14)*u(4)*u(17)-u(16)^2*u(8)*u(14)*u(4)*u(7)-u(16)*u(8)*u(12)*u(1)*u(11)*u(3)-u(16)*u(8)*u(12)*u(1)*u(14)*u(6)-u(16)*u(8)*u(12)*u(1)*u(17)*u(9)-u(16)*u(8)*u(15)*u(4)*u(11)*u(3)-u(16)*u(8)*u(15)*u(4)*u(14)*u(6)-u(16)*u(8)*u(15)*u(4)*u(17)*u(9)-u(16)*u(8)*u(18)*u(7)*u(11)*u(3)-u(16)*u(8)*u(18)*u(7)*u(14)*u(6)-u(10)*u(3)*u(15)^2*u(4)*u(6)-u(10)*u(3)*u(15)*u(4)^2*u(13)-u(10)*u(3)*u(18)^2*u(7)*u(9)-u(10)*u(3)*u(18)*u(7)^2*u(16)-u(10)*u(3)*u(11)*u(1)*u(15)*u(5)-u(10)*u(3)*u(11)*u(1)*u(18)*u(8)-u(10)*u(3)*u(14)*u(4)*u(12)*u(2)-u(10)*u(3)*u(14)*u(4)*u(15)*u(5)-u(10)*u(3)*u(14)*u(4)*u(18)*u(8)-u(10)*u(3)*u(17)*u(7)*u(12)*u(2)-u(10)*u(3)*u(17)*u(7)*u(15)*u(5)-u(10)*u(3)*u(17)*u(7)*u(18)*u(8)-u(10)*u(3)^2*u(15)*u(4)*u(12)-u(10)^2*u(3)*u(15)*u(4)*u(1)-u(10)*u(3)*u(15)*u(4)*u(18)*u(9)-u(10)*u(3)*u(15)*u(4)*u(16)*u(7)-u(10)*u(3)^2*u(18)*u(7)*u(12)-u(10)^2*u(3)*u(18)*u(7)*u(1)-u(10)*u(3)*u(18)*u(7)*u(15)*u(6)-u(10)*u(3)*u(18)*u(7)*u(13)*u(4)-u(13)*u(6)*u(12)*u(1)^2*u(10)-u(13)*u(6)*u(12)^2*u(1)*u(3)-u(13)*u(6)*u(18)^2*u(7)*u(9)-u(13)*u(6)*u(18)*u(7)^2*u(16)-u(13)*u(6)*u(11)*u(1)*u(12)*u(2)-u(13)*u(6)*u(11)*u(1)*u(15)*u(5)-u(13)*u(6)*u(11)*u(1)*u(18)*u(8)-u(13)*u(6)*u(14)*u(4)*u(12)*u(2)-u(13)*u(6)*u(14)*u(4)*u(18)*u(8)-u(13)*u(6)*u(17)*u(7)*u(12)*u(2)-u(13)*u(6)*u(17)*u(7)*u(15)*u(5)-u(13)*u(6)*u(17)*u(7)*u(18)*u(8)-u(13)*u(6)^2*u(12)*u(1)*u(15)-u(13)^2*u(6)*u(12)*u(1)*u(4)-u(13)*u(6)*u(12)*u(1)*u(18)*u(9)-u(13)*u(6)*u(12)*u(1)*u(16)*u(7)-u(13)*u(6)*u(18)*u(7)*u(12)*u(3)-u(13)*u(6)*u(18)*u(7)*u(10)*u(1)-u(13)*u(6)^2*u(18)*u(7)*u(15)-u(13)^2*u(6)*u(18)*u(7)*u(4)-u(16)*u(9)*u(12)*u(1)^2*u(10)-u(16)*u(9)*u(12)^2*u(1)*u(3)-u(16)*u(9)*u(15)^2*u(4)*u(6)-u(16)*u(9)*u(15)*u(4)^2*u(13)-u(16)*u(9)*u(11)*u(1)*u(12)*u(2)-u(16)*u(9)*u(11)*u(1)*u(15)*u(5)-u(16)*u(9)*u(11)*u(1)*u(18)*u(8)-u(16)*u(9)*u(14)*u(4)*u(12)*u(2)-u(16)*u(9)*u(14)*u(4)*u(15)*u(5)-u(16)*u(9)*u(14)*u(4)*u(18)*u(8)-u(16)*u(9)*u(17)*u(7)*u(12)*u(2)-u(16)*u(9)*u(17)*u(7)*u(15)*u(5)-u(16)*u(9)*u(12)*u(1)*u(15)*u(6)-u(16)*u(9)*u(12)*u(1)*u(13)*u(4)-u(16)*u(9)^2*u(12)*u(1)*u(18)-u(16)^2*u(9)*u(12)*u(1)*u(7)-u(16)*u(9)*u(15)*u(4)*u(12)*u(3)-u(16)*u(9)*u(15)*u(4)*u(10)*u(1)-u(16)*u(9)^2*u(15)*u(4)*u(18)-u(16)^2*u(9)*u(15)*u(4)*u(7))*u(19)+2*(u(12)*u(3)^2*u(11)+u(14)^2*u(5)*u(6)+u(11)^2*u(2)*u(3)+u(18)*u(9)^2*u(17)+u(15)*u(6)^2*u(14)+u(17)^2*u(8)*u(9)+u(12)*u(3)*u(14)*u(6)+u(12)*u(3)*u(17)*u(9)+u(11)*u(2)*u(14)*u(6)+u(11)*u(2)*u(17)*u(9)+u(15)*u(6)*u(11)*u(3)+u(15)*u(6)*u(17)*u(9)+u(14)*u(5)*u(11)*u(3)+u(14)*u(5)*u(17)*u(9)+u(18)*u(9)*u(11)*u(3)+u(18)*u(9)*u(14)*u(6)+u(17)*u(8)*u(11)*u(3)+u(17)*u(8)*u(14)*u(6)+u(11)*u(1)*u(10)*u(3)+u(11)*u(1)*u(13)*u(6)+u(11)*u(1)*u(16)*u(9)+u(14)*u(4)*u(10)*u(3)+u(14)*u(4)*u(13)*u(6)+u(14)*u(4)*u(16)*u(9)+u(17)*u(7)*u(10)*u(3)+u(17)*u(7)*u(13)*u(6)+u(17)*u(7)*u(16)*u(9))/(u(12)*u(3)*u(13)^2*u(4)^2+u(12)*u(3)*u(16)^2*u(7)^2+u(12)^2*u(3)^2*u(14)*u(5)+u(12)^2*u(3)^2*u(13)*u(4)+u(12)^2*u(3)^2*u(17)*u(8)+u(12)^2*u(3)^2*u(16)*u(7)+u(11)*u(2)*u(13)^2*u(4)^2+u(11)*u(2)*u(16)^2*u(7)^2+u(11)^2*u(2)^2*u(15)*u(6)+u(11)^2*u(2)^2*u(13)*u(4)+u(11)^2*u(2)^2*u(18)*u(9)+u(11)^2*u(2)^2*u(16)*u(7)+u(15)*u(6)*u(10)^2*u(1)^2+u(15)*u(6)*u(16)^2*u(7)^2+u(15)^2*u(6)^2*u(11)*u(2)+u(15)^2*u(6)^2*u(10)*u(1)+u(15)^2*u(6)^2*u(17)*u(8)+u(15)^2*u(6)^2*u(16)*u(7)+u(14)*u(5)*u(10)^2*u(1)^2+u(14)*u(5)*u(16)^2*u(7)^2+u(14)^2*u(5)^2*u(12)*u(3)+u(14)^2*u(5)^2*u(10)*u(1)+u(14)^2*u(5)^2*u(18)*u(9)+u(14)^2*u(5)^2*u(16)*u(7)+u(18)*u(9)*u(10)^2*u(1)^2+u(18)*u(9)*u(13)^2*u(4)^2+u(18)^2*u(9)^2*u(11)*u(2)+u(18)^2*u(9)^2*u(10)*u(1)+u(18)^2*u(9)^2*u(14)*u(5)+u(18)^2*u(9)^2*u(13)*u(4)+u(17)*u(8)*u(10)^2*u(1)^2+u(17)*u(8)*u(13)^2*u(4)^2+u(17)^2*u(8)^2*u(12)*u(3)+u(17)^2*u(8)^2*u(10)*u(1)+u(17)^2*u(8)^2*u(15)*u(6)+u(17)^2*u(8)^2*u(13)*u(4)-u(10)*u(2)*u(14)^2*u(4)*u(5)-u(10)*u(2)*u(14)*u(4)^2*u(13)-u(10)*u(2)*u(17)*u(7)^2*u(16)-u(10)*u(2)*u(17)^2*u(7)*u(8)-u(10)*u(2)^2*u(14)*u(4)*u(11)+2*u(12)*u(3)*u(10)*u(1)*u(14)*u(5)+u(12)*u(3)*u(10)*u(1)*u(13)*u(4)+2*u(12)*u(3)*u(10)*u(1)*u(17)*u(8)+u(12)*u(3)*u(10)*u(1)*u(16)*u(7)+u(12)*u(3)*u(15)*u(6)*u(11)*u(2)+u(12)*u(3)*u(15)*u(6)*u(10)*u(1)+u(12)*u(3)*u(15)*u(6)*u(13)*u(4)+2*u(12)*u(3)*u(15)*u(6)*u(17)*u(8)+2*u(12)*u(3)*u(15)*u(6)*u(16)*u(7)+2*u(12)*u(3)*u(13)*u(4)*u(11)*u(2)+2*u(12)*u(3)*u(13)*u(4)*u(14)*u(5)+2*u(12)*u(3)*u(13)*u(4)*u(17)*u(8)+2*u(12)*u(3)*u(13)*u(4)*u(16)*u(7)+u(12)*u(3)*u(18)*u(9)*u(11)*u(2)+u(12)*u(3)*u(18)*u(9)*u(10)*u(1)+2*u(12)*u(3)*u(18)*u(9)*u(14)*u(5)+2*u(12)*u(3)*u(18)*u(9)*u(13)*u(4)+u(12)*u(3)*u(18)*u(9)*u(16)*u(7)+2*u(12)*u(3)*u(16)*u(7)*u(11)*u(2)+2*u(12)*u(3)*u(16)*u(7)*u(14)*u(5)+2*u(12)*u(3)*u(16)*u(7)*u(17)*u(8)-u(12)^2*u(3)*u(2)*u(14)*u(6)-u(12)^2*u(3)*u(2)*u(17)*u(9)-u(12)*u(3)^2*u(15)*u(5)*u(11)-u(12)*u(3)*u(15)*u(5)*u(17)*u(9)-u(12)*u(3)^2*u(18)*u(8)*u(11)-u(12)*u(3)*u(18)*u(8)*u(14)*u(6)+u(11)*u(2)*u(12)*u(3)*u(14)*u(5)+u(11)*u(2)*u(12)*u(3)*u(17)*u(8)+u(11)*u(2)*u(10)*u(1)*u(14)*u(5)+u(11)*u(2)*u(10)*u(1)*u(13)*u(4)+u(11)*u(2)*u(10)*u(1)*u(17)*u(8)+u(11)*u(2)*u(10)*u(1)*u(16)*u(7)+2*u(11)*u(2)*u(15)*u(6)*u(10)*u(1)+2*u(11)*u(2)*u(15)*u(6)*u(13)*u(4)+2*u(11)*u(2)*u(15)*u(6)*u(17)*u(8)+2*u(11)*u(2)*u(15)*u(6)*u(16)*u(7)+u(11)*u(2)*u(13)*u(4)*u(14)*u(5)+2*u(11)*u(2)*u(13)*u(4)*u(17)*u(8)+2*u(11)*u(2)*u(13)*u(4)*u(16)*u(7)+2*u(11)*u(2)*u(18)*u(9)*u(10)*u(1)+2*u(11)*u(2)*u(18)*u(9)*u(14)*u(5)+2*u(11)*u(2)*u(18)*u(9)*u(13)*u(4)+2*u(11)*u(2)*u(18)*u(9)*u(16)*u(7)+2*u(11)*u(2)*u(16)*u(7)*u(14)*u(5)+u(11)*u(2)*u(16)*u(7)*u(17)*u(8)-u(11)*u(2)^2*u(12)*u(14)*u(6)-u(11)*u(2)^2*u(12)*u(17)*u(9)-u(11)^2*u(2)*u(15)*u(5)*u(3)-u(11)*u(2)*u(15)*u(5)*u(17)*u(9)-u(11)^2*u(2)*u(18)*u(8)*u(3)-u(11)*u(2)*u(18)*u(8)*u(14)*u(6)+u(15)*u(6)*u(12)*u(3)*u(14)*u(5)+2*u(15)*u(6)*u(10)*u(1)*u(14)*u(5)+u(15)*u(6)*u(10)*u(1)*u(13)*u(4)+2*u(15)*u(6)*u(10)*u(1)*u(17)*u(8)+2*u(15)*u(6)*u(10)*u(1)*u(16)*u(7)+2*u(15)*u(6)*u(13)*u(4)*u(17)*u(8)+u(15)*u(6)*u(13)*u(4)*u(16)*u(7)+2*u(15)*u(6)*u(18)*u(9)*u(11)*u(2)+2*u(15)*u(6)*u(18)*u(9)*u(10)*u(1)+u(15)*u(6)*u(18)*u(9)*u(14)*u(5)+u(15)*u(6)*u(18)*u(9)*u(13)*u(4)+u(15)*u(6)*u(18)*u(9)*u(16)*u(7)+2*u(15)*u(6)*u(16)*u(7)*u(14)*u(5)+2*u(15)*u(6)*u(16)*u(7)*u(17)*u(8)-u(15)*u(6)^2*u(12)*u(2)*u(14)-u(15)*u(6)*u(12)*u(2)*u(17)*u(9)-u(15)^2*u(6)*u(5)*u(11)*u(3)-u(15)^2*u(6)*u(5)*u(17)*u(9)-u(15)*u(6)*u(18)*u(8)*u(11)*u(3)-u(15)*u(6)^2*u(18)*u(8)*u(14)+2*u(14)*u(5)*u(12)*u(3)*u(17)*u(8)+u(14)*u(5)*u(10)*u(1)*u(13)*u(4)+2*u(14)*u(5)*u(10)*u(1)*u(17)*u(8)+2*u(14)*u(5)*u(10)*u(1)*u(16)*u(7)+u(14)*u(5)*u(15)*u(6)*u(11)*u(2)+u(14)*u(5)*u(15)*u(6)*u(17)*u(8)+u(14)*u(5)*u(13)*u(4)*u(17)*u(8)+u(14)*u(5)*u(13)*u(4)*u(16)*u(7)+2*u(14)*u(5)*u(18)*u(9)*u(10)*u(1)+2*u(14)*u(5)*u(18)*u(9)*u(13)*u(4)+2*u(14)*u(5)*u(18)*u(9)*u(16)*u(7)+u(14)*u(5)*u(16)*u(7)*u(17)*u(8)-u(14)^2*u(5)*u(12)*u(2)*u(6)-u(14)*u(5)*u(12)*u(2)*u(17)*u(9)-u(14)*u(5)^2*u(15)*u(11)*u(3)-u(14)*u(5)^2*u(15)*u(17)*u(9)-u(14)*u(5)*u(18)*u(8)*u(11)*u(3)-u(14)^2*u(5)*u(18)*u(8)*u(6)+u(18)*u(9)*u(12)*u(3)*u(17)*u(8)+2*u(18)*u(9)*u(10)*u(1)*u(13)*u(4)+2*u(18)*u(9)*u(10)*u(1)*u(17)*u(8)+u(18)*u(9)*u(10)*u(1)*u(16)*u(7)+u(18)*u(9)*u(15)*u(6)*u(17)*u(8)+2*u(18)*u(9)*u(13)*u(4)*u(17)*u(8)+u(18)*u(9)*u(13)*u(4)*u(16)*u(7)-u(18)*u(9)*u(12)*u(2)*u(14)*u(6)-u(18)*u(9)^2*u(12)*u(2)*u(17)-u(18)*u(9)*u(15)*u(5)*u(11)*u(3)-u(18)*u(9)^2*u(15)*u(5)*u(17)-u(18)^2*u(9)*u(8)*u(11)*u(3)-u(18)^2*u(9)*u(8)*u(14)*u(6)+2*u(17)*u(8)*u(10)*u(1)*u(13)*u(4)+u(17)*u(8)*u(10)*u(1)*u(16)*u(7)+u(17)*u(8)*u(13)*u(4)*u(16)*u(7)+u(17)*u(8)*u(18)*u(9)*u(11)*u(2)+u(17)*u(8)*u(18)*u(9)*u(14)*u(5)-u(17)*u(8)*u(12)*u(2)*u(14)*u(6)-u(17)^2*u(8)*u(12)*u(2)*u(9)-u(17)*u(8)*u(15)*u(5)*u(11)*u(3)-u(17)^2*u(8)*u(15)*u(5)*u(9)-u(17)*u(8)^2*u(18)*u(11)*u(3)-u(17)*u(8)^2*u(18)*u(14)*u(6)-u(10)^2*u(2)*u(14)*u(4)*u(1)-u(10)*u(2)*u(14)*u(4)*u(17)*u(8)-u(10)*u(2)*u(14)*u(4)*u(16)*u(7)-u(10)*u(2)^2*u(17)*u(7)*u(11)-u(10)^2*u(2)*u(17)*u(7)*u(1)-u(10)*u(2)*u(17)*u(7)*u(14)*u(5)-u(10)*u(2)*u(17)*u(7)*u(13)*u(4)-u(10)*u(2)*u(12)*u(1)*u(14)*u(6)-u(10)*u(2)*u(12)*u(1)*u(17)*u(9)-u(10)*u(2)*u(15)*u(4)*u(11)*u(3)-u(10)*u(2)*u(15)*u(4)*u(14)*u(6)-u(10)*u(2)*u(15)*u(4)*u(17)*u(9)-u(10)*u(2)*u(18)*u(7)*u(11)*u(3)-u(10)*u(2)*u(18)*u(7)*u(14)*u(6)-u(10)*u(2)*u(18)*u(7)*u(17)*u(9)-u(13)*u(5)*u(11)^2*u(1)*u(2)-u(13)*u(5)*u(11)*u(1)^2*u(10)-u(13)*u(5)*u(17)*u(7)^2*u(16)-u(13)*u(5)*u(17)^2*u(7)*u(8)-u(13)*u(5)^2*u(11)*u(1)*u(14)-u(13)^2*u(5)*u(11)*u(1)*u(4)-u(13)*u(5)*u(11)*u(1)*u(17)*u(8)-u(13)*u(5)*u(11)*u(1)*u(16)*u(7)-u(13)*u(5)*u(17)*u(7)*u(11)*u(2)-u(13)*u(5)*u(17)*u(7)*u(10)*u(1)-u(13)*u(5)^2*u(17)*u(7)*u(14)-u(13)^2*u(5)*u(17)*u(7)*u(4)-u(13)*u(5)*u(12)*u(1)*u(11)*u(3)-u(13)*u(5)*u(12)*u(1)*u(14)*u(6)-u(13)*u(5)*u(12)*u(1)*u(17)*u(9)-u(13)*u(5)*u(15)*u(4)*u(11)*u(3)-u(13)*u(5)*u(15)*u(4)*u(17)*u(9)-u(13)*u(5)*u(18)*u(7)*u(11)*u(3)-u(13)*u(5)*u(18)*u(7)*u(14)*u(6)-u(13)*u(5)*u(18)*u(7)*u(17)*u(9)-u(16)*u(8)*u(14)^2*u(4)*u(5)-u(16)*u(8)*u(11)^2*u(1)*u(2)-u(16)*u(8)*u(14)*u(4)^2*u(13)-u(16)*u(8)*u(11)*u(1)^2*u(10)-u(16)*u(8)*u(11)*u(1)*u(14)*u(5)-u(16)*u(8)*u(11)*u(1)*u(13)*u(4)-u(16)*u(8)^2*u(11)*u(1)*u(17)-u(16)^2*u(8)*u(11)*u(1)*u(7)-u(16)*u(8)*u(14)*u(4)*u(11)*u(2)-u(16)*u(8)*u(14)*u(4)*u(10)*u(1)-u(16)*u(8)^2*u(14)*u(4)*u(17)-u(16)^2*u(8)*u(14)*u(4)*u(7)-u(16)*u(8)*u(12)*u(1)*u(11)*u(3)-u(16)*u(8)*u(12)*u(1)*u(14)*u(6)-u(16)*u(8)*u(12)*u(1)*u(17)*u(9)-u(16)*u(8)*u(15)*u(4)*u(11)*u(3)-u(16)*u(8)*u(15)*u(4)*u(14)*u(6)-u(16)*u(8)*u(15)*u(4)*u(17)*u(9)-u(16)*u(8)*u(18)*u(7)*u(11)*u(3)-u(16)*u(8)*u(18)*u(7)*u(14)*u(6)-u(10)*u(3)*u(15)^2*u(4)*u(6)-u(10)*u(3)*u(15)*u(4)^2*u(13)-u(10)*u(3)*u(18)^2*u(7)*u(9)-u(10)*u(3)*u(18)*u(7)^2*u(16)-u(10)*u(3)*u(11)*u(1)*u(15)*u(5)-u(10)*u(3)*u(11)*u(1)*u(18)*u(8)-u(10)*u(3)*u(14)*u(4)*u(12)*u(2)-u(10)*u(3)*u(14)*u(4)*u(15)*u(5)-u(10)*u(3)*u(14)*u(4)*u(18)*u(8)-u(10)*u(3)*u(17)*u(7)*u(12)*u(2)-u(10)*u(3)*u(17)*u(7)*u(15)*u(5)-u(10)*u(3)*u(17)*u(7)*u(18)*u(8)-u(10)*u(3)^2*u(15)*u(4)*u(12)-u(10)^2*u(3)*u(15)*u(4)*u(1)-u(10)*u(3)*u(15)*u(4)*u(18)*u(9)-u(10)*u(3)*u(15)*u(4)*u(16)*u(7)-u(10)*u(3)^2*u(18)*u(7)*u(12)-u(10)^2*u(3)*u(18)*u(7)*u(1)-u(10)*u(3)*u(18)*u(7)*u(15)*u(6)-u(10)*u(3)*u(18)*u(7)*u(13)*u(4)-u(13)*u(6)*u(12)*u(1)^2*u(10)-u(13)*u(6)*u(12)^2*u(1)*u(3)-u(13)*u(6)*u(18)^2*u(7)*u(9)-u(13)*u(6)*u(18)*u(7)^2*u(16)-u(13)*u(6)*u(11)*u(1)*u(12)*u(2)-u(13)*u(6)*u(11)*u(1)*u(15)*u(5)-u(13)*u(6)*u(11)*u(1)*u(18)*u(8)-u(13)*u(6)*u(14)*u(4)*u(12)*u(2)-u(13)*u(6)*u(14)*u(4)*u(18)*u(8)-u(13)*u(6)*u(17)*u(7)*u(12)*u(2)-u(13)*u(6)*u(17)*u(7)*u(15)*u(5)-u(13)*u(6)*u(17)*u(7)*u(18)*u(8)-u(13)*u(6)^2*u(12)*u(1)*u(15)-u(13)^2*u(6)*u(12)*u(1)*u(4)-u(13)*u(6)*u(12)*u(1)*u(18)*u(9)-u(13)*u(6)*u(12)*u(1)*u(16)*u(7)-u(13)*u(6)*u(18)*u(7)*u(12)*u(3)-u(13)*u(6)*u(18)*u(7)*u(10)*u(1)-u(13)*u(6)^2*u(18)*u(7)*u(15)-u(13)^2*u(6)*u(18)*u(7)*u(4)-u(16)*u(9)*u(12)*u(1)^2*u(10)-u(16)*u(9)*u(12)^2*u(1)*u(3)-u(16)*u(9)*u(15)^2*u(4)*u(6)-u(16)*u(9)*u(15)*u(4)^2*u(13)-u(16)*u(9)*u(11)*u(1)*u(12)*u(2)-u(16)*u(9)*u(11)*u(1)*u(15)*u(5)-u(16)*u(9)*u(11)*u(1)*u(18)*u(8)-u(16)*u(9)*u(14)*u(4)*u(12)*u(2)-u(16)*u(9)*u(14)*u(4)*u(15)*u(5)-u(16)*u(9)*u(14)*u(4)*u(18)*u(8)-u(16)*u(9)*u(17)*u(7)*u(12)*u(2)-u(16)*u(9)*u(17)*u(7)*u(15)*u(5)-u(16)*u(9)*u(12)*u(1)*u(15)*u(6)-u(16)*u(9)*u(12)*u(1)*u(13)*u(4)-u(16)*u(9)^2*u(12)*u(1)*u(18)-u(16)^2*u(9)*u(12)*u(1)*u(7)-u(16)*u(9)*u(15)*u(4)*u(12)*u(3)-u(16)*u(9)*u(15)*u(4)*u(10)*u(1)-u(16)*u(9)^2*u(15)*u(4)*u(18)-u(16)^2*u(9)*u(15)*u(4)*u(7))*u(20)+2*(u(12)*u(3)*u(11)*u(2)+u(12)*u(3)*u(10)*u(1)+u(12)*u(3)*u(14)*u(5)+u(12)*u(3)*u(13)*u(4)+u(12)*u(3)*u(17)*u(8)+u(12)*u(3)*u(16)*u(7)+u(10)*u(1)*u(14)*u(5)+u(10)*u(1)*u(17)*u(8)+u(15)*u(6)*u(11)*u(2)+u(15)*u(6)*u(10)*u(1)+u(15)*u(6)*u(14)*u(5)+u(15)*u(6)*u(13)*u(4)+u(15)*u(6)*u(17)*u(8)+u(15)*u(6)*u(16)*u(7)+u(13)*u(4)*u(11)*u(2)+u(13)*u(4)*u(17)*u(8)+u(18)*u(9)*u(11)*u(2)+u(18)*u(9)*u(10)*u(1)+u(18)*u(9)*u(14)*u(5)+u(18)*u(9)*u(13)*u(4)+u(18)*u(9)*u(17)*u(8)+u(18)*u(9)*u(16)*u(7)+u(16)*u(7)*u(11)*u(2)+u(16)*u(7)*u(14)*u(5)+2*u(12)*u(3)*u(15)*u(6)+2*u(12)*u(3)*u(18)*u(9)+2*u(15)*u(6)*u(18)*u(9)-u(11)*u(1)*u(13)*u(5)-u(11)*u(1)*u(16)*u(8)-u(14)*u(4)*u(10)*u(2)-u(14)*u(4)*u(16)*u(8)-u(17)*u(7)*u(10)*u(2)+u(12)^2*u(3)^2+u(15)^2*u(6)^2+u(18)^2*u(9)^2-u(17)*u(7)*u(13)*u(5))/(u(12)*u(3)*u(13)^2*u(4)^2+u(12)*u(3)*u(16)^2*u(7)^2+u(12)^2*u(3)^2*u(14)*u(5)+u(12)^2*u(3)^2*u(13)*u(4)+u(12)^2*u(3)^2*u(17)*u(8)+u(12)^2*u(3)^2*u(16)*u(7)+u(11)*u(2)*u(13)^2*u(4)^2+u(11)*u(2)*u(16)^2*u(7)^2+u(11)^2*u(2)^2*u(15)*u(6)+u(11)^2*u(2)^2*u(13)*u(4)+u(11)^2*u(2)^2*u(18)*u(9)+u(11)^2*u(2)^2*u(16)*u(7)+u(15)*u(6)*u(10)^2*u(1)^2+u(15)*u(6)*u(16)^2*u(7)^2+u(15)^2*u(6)^2*u(11)*u(2)+u(15)^2*u(6)^2*u(10)*u(1)+u(15)^2*u(6)^2*u(17)*u(8)+u(15)^2*u(6)^2*u(16)*u(7)+u(14)*u(5)*u(10)^2*u(1)^2+u(14)*u(5)*u(16)^2*u(7)^2+u(14)^2*u(5)^2*u(12)*u(3)+u(14)^2*u(5)^2*u(10)*u(1)+u(14)^2*u(5)^2*u(18)*u(9)+u(14)^2*u(5)^2*u(16)*u(7)+u(18)*u(9)*u(10)^2*u(1)^2+u(18)*u(9)*u(13)^2*u(4)^2+u(18)^2*u(9)^2*u(11)*u(2)+u(18)^2*u(9)^2*u(10)*u(1)+u(18)^2*u(9)^2*u(14)*u(5)+u(18)^2*u(9)^2*u(13)*u(4)+u(17)*u(8)*u(10)^2*u(1)^2+u(17)*u(8)*u(13)^2*u(4)^2+u(17)^2*u(8)^2*u(12)*u(3)+u(17)^2*u(8)^2*u(10)*u(1)+u(17)^2*u(8)^2*u(15)*u(6)+u(17)^2*u(8)^2*u(13)*u(4)-u(10)*u(2)*u(14)^2*u(4)*u(5)-u(10)*u(2)*u(14)*u(4)^2*u(13)-u(10)*u(2)*u(17)*u(7)^2*u(16)-u(10)*u(2)*u(17)^2*u(7)*u(8)-u(10)*u(2)^2*u(14)*u(4)*u(11)+2*u(12)*u(3)*u(10)*u(1)*u(14)*u(5)+u(12)*u(3)*u(10)*u(1)*u(13)*u(4)+2*u(12)*u(3)*u(10)*u(1)*u(17)*u(8)+u(12)*u(3)*u(10)*u(1)*u(16)*u(7)+u(12)*u(3)*u(15)*u(6)*u(11)*u(2)+u(12)*u(3)*u(15)*u(6)*u(10)*u(1)+u(12)*u(3)*u(15)*u(6)*u(13)*u(4)+2*u(12)*u(3)*u(15)*u(6)*u(17)*u(8)+2*u(12)*u(3)*u(15)*u(6)*u(16)*u(7)+2*u(12)*u(3)*u(13)*u(4)*u(11)*u(2)+2*u(12)*u(3)*u(13)*u(4)*u(14)*u(5)+2*u(12)*u(3)*u(13)*u(4)*u(17)*u(8)+2*u(12)*u(3)*u(13)*u(4)*u(16)*u(7)+u(12)*u(3)*u(18)*u(9)*u(11)*u(2)+u(12)*u(3)*u(18)*u(9)*u(10)*u(1)+2*u(12)*u(3)*u(18)*u(9)*u(14)*u(5)+2*u(12)*u(3)*u(18)*u(9)*u(13)*u(4)+u(12)*u(3)*u(18)*u(9)*u(16)*u(7)+2*u(12)*u(3)*u(16)*u(7)*u(11)*u(2)+2*u(12)*u(3)*u(16)*u(7)*u(14)*u(5)+2*u(12)*u(3)*u(16)*u(7)*u(17)*u(8)-u(12)^2*u(3)*u(2)*u(14)*u(6)-u(12)^2*u(3)*u(2)*u(17)*u(9)-u(12)*u(3)^2*u(15)*u(5)*u(11)-u(12)*u(3)*u(15)*u(5)*u(17)*u(9)-u(12)*u(3)^2*u(18)*u(8)*u(11)-u(12)*u(3)*u(18)*u(8)*u(14)*u(6)+u(11)*u(2)*u(12)*u(3)*u(14)*u(5)+u(11)*u(2)*u(12)*u(3)*u(17)*u(8)+u(11)*u(2)*u(10)*u(1)*u(14)*u(5)+u(11)*u(2)*u(10)*u(1)*u(13)*u(4)+u(11)*u(2)*u(10)*u(1)*u(17)*u(8)+u(11)*u(2)*u(10)*u(1)*u(16)*u(7)+2*u(11)*u(2)*u(15)*u(6)*u(10)*u(1)+2*u(11)*u(2)*u(15)*u(6)*u(13)*u(4)+2*u(11)*u(2)*u(15)*u(6)*u(17)*u(8)+2*u(11)*u(2)*u(15)*u(6)*u(16)*u(7)+u(11)*u(2)*u(13)*u(4)*u(14)*u(5)+2*u(11)*u(2)*u(13)*u(4)*u(17)*u(8)+2*u(11)*u(2)*u(13)*u(4)*u(16)*u(7)+2*u(11)*u(2)*u(18)*u(9)*u(10)*u(1)+2*u(11)*u(2)*u(18)*u(9)*u(14)*u(5)+2*u(11)*u(2)*u(18)*u(9)*u(13)*u(4)+2*u(11)*u(2)*u(18)*u(9)*u(16)*u(7)+2*u(11)*u(2)*u(16)*u(7)*u(14)*u(5)+u(11)*u(2)*u(16)*u(7)*u(17)*u(8)-u(11)*u(2)^2*u(12)*u(14)*u(6)-u(11)*u(2)^2*u(12)*u(17)*u(9)-u(11)^2*u(2)*u(15)*u(5)*u(3)-u(11)*u(2)*u(15)*u(5)*u(17)*u(9)-u(11)^2*u(2)*u(18)*u(8)*u(3)-u(11)*u(2)*u(18)*u(8)*u(14)*u(6)+u(15)*u(6)*u(12)*u(3)*u(14)*u(5)+2*u(15)*u(6)*u(10)*u(1)*u(14)*u(5)+u(15)*u(6)*u(10)*u(1)*u(13)*u(4)+2*u(15)*u(6)*u(10)*u(1)*u(17)*u(8)+2*u(15)*u(6)*u(10)*u(1)*u(16)*u(7)+2*u(15)*u(6)*u(13)*u(4)*u(17)*u(8)+u(15)*u(6)*u(13)*u(4)*u(16)*u(7)+2*u(15)*u(6)*u(18)*u(9)*u(11)*u(2)+2*u(15)*u(6)*u(18)*u(9)*u(10)*u(1)+u(15)*u(6)*u(18)*u(9)*u(14)*u(5)+u(15)*u(6)*u(18)*u(9)*u(13)*u(4)+u(15)*u(6)*u(18)*u(9)*u(16)*u(7)+2*u(15)*u(6)*u(16)*u(7)*u(14)*u(5)+2*u(15)*u(6)*u(16)*u(7)*u(17)*u(8)-u(15)*u(6)^2*u(12)*u(2)*u(14)-u(15)*u(6)*u(12)*u(2)*u(17)*u(9)-u(15)^2*u(6)*u(5)*u(11)*u(3)-u(15)^2*u(6)*u(5)*u(17)*u(9)-u(15)*u(6)*u(18)*u(8)*u(11)*u(3)-u(15)*u(6)^2*u(18)*u(8)*u(14)+2*u(14)*u(5)*u(12)*u(3)*u(17)*u(8)+u(14)*u(5)*u(10)*u(1)*u(13)*u(4)+2*u(14)*u(5)*u(10)*u(1)*u(17)*u(8)+2*u(14)*u(5)*u(10)*u(1)*u(16)*u(7)+u(14)*u(5)*u(15)*u(6)*u(11)*u(2)+u(14)*u(5)*u(15)*u(6)*u(17)*u(8)+u(14)*u(5)*u(13)*u(4)*u(17)*u(8)+u(14)*u(5)*u(13)*u(4)*u(16)*u(7)+2*u(14)*u(5)*u(18)*u(9)*u(10)*u(1)+2*u(14)*u(5)*u(18)*u(9)*u(13)*u(4)+2*u(14)*u(5)*u(18)*u(9)*u(16)*u(7)+u(14)*u(5)*u(16)*u(7)*u(17)*u(8)-u(14)^2*u(5)*u(12)*u(2)*u(6)-u(14)*u(5)*u(12)*u(2)*u(17)*u(9)-u(14)*u(5)^2*u(15)*u(11)*u(3)-u(14)*u(5)^2*u(15)*u(17)*u(9)-u(14)*u(5)*u(18)*u(8)*u(11)*u(3)-u(14)^2*u(5)*u(18)*u(8)*u(6)+u(18)*u(9)*u(12)*u(3)*u(17)*u(8)+2*u(18)*u(9)*u(10)*u(1)*u(13)*u(4)+2*u(18)*u(9)*u(10)*u(1)*u(17)*u(8)+u(18)*u(9)*u(10)*u(1)*u(16)*u(7)+u(18)*u(9)*u(15)*u(6)*u(17)*u(8)+2*u(18)*u(9)*u(13)*u(4)*u(17)*u(8)+u(18)*u(9)*u(13)*u(4)*u(16)*u(7)-u(18)*u(9)*u(12)*u(2)*u(14)*u(6)-u(18)*u(9)^2*u(12)*u(2)*u(17)-u(18)*u(9)*u(15)*u(5)*u(11)*u(3)-u(18)*u(9)^2*u(15)*u(5)*u(17)-u(18)^2*u(9)*u(8)*u(11)*u(3)-u(18)^2*u(9)*u(8)*u(14)*u(6)+2*u(17)*u(8)*u(10)*u(1)*u(13)*u(4)+u(17)*u(8)*u(10)*u(1)*u(16)*u(7)+u(17)*u(8)*u(13)*u(4)*u(16)*u(7)+u(17)*u(8)*u(18)*u(9)*u(11)*u(2)+u(17)*u(8)*u(18)*u(9)*u(14)*u(5)-u(17)*u(8)*u(12)*u(2)*u(14)*u(6)-u(17)^2*u(8)*u(12)*u(2)*u(9)-u(17)*u(8)*u(15)*u(5)*u(11)*u(3)-u(17)^2*u(8)*u(15)*u(5)*u(9)-u(17)*u(8)^2*u(18)*u(11)*u(3)-u(17)*u(8)^2*u(18)*u(14)*u(6)-u(10)^2*u(2)*u(14)*u(4)*u(1)-u(10)*u(2)*u(14)*u(4)*u(17)*u(8)-u(10)*u(2)*u(14)*u(4)*u(16)*u(7)-u(10)*u(2)^2*u(17)*u(7)*u(11)-u(10)^2*u(2)*u(17)*u(7)*u(1)-u(10)*u(2)*u(17)*u(7)*u(14)*u(5)-u(10)*u(2)*u(17)*u(7)*u(13)*u(4)-u(10)*u(2)*u(12)*u(1)*u(14)*u(6)-u(10)*u(2)*u(12)*u(1)*u(17)*u(9)-u(10)*u(2)*u(15)*u(4)*u(11)*u(3)-u(10)*u(2)*u(15)*u(4)*u(14)*u(6)-u(10)*u(2)*u(15)*u(4)*u(17)*u(9)-u(10)*u(2)*u(18)*u(7)*u(11)*u(3)-u(10)*u(2)*u(18)*u(7)*u(14)*u(6)-u(10)*u(2)*u(18)*u(7)*u(17)*u(9)-u(13)*u(5)*u(11)^2*u(1)*u(2)-u(13)*u(5)*u(11)*u(1)^2*u(10)-u(13)*u(5)*u(17)*u(7)^2*u(16)-u(13)*u(5)*u(17)^2*u(7)*u(8)-u(13)*u(5)^2*u(11)*u(1)*u(14)-u(13)^2*u(5)*u(11)*u(1)*u(4)-u(13)*u(5)*u(11)*u(1)*u(17)*u(8)-u(13)*u(5)*u(11)*u(1)*u(16)*u(7)-u(13)*u(5)*u(17)*u(7)*u(11)*u(2)-u(13)*u(5)*u(17)*u(7)*u(10)*u(1)-u(13)*u(5)^2*u(17)*u(7)*u(14)-u(13)^2*u(5)*u(17)*u(7)*u(4)-u(13)*u(5)*u(12)*u(1)*u(11)*u(3)-u(13)*u(5)*u(12)*u(1)*u(14)*u(6)-u(13)*u(5)*u(12)*u(1)*u(17)*u(9)-u(13)*u(5)*u(15)*u(4)*u(11)*u(3)-u(13)*u(5)*u(15)*u(4)*u(17)*u(9)-u(13)*u(5)*u(18)*u(7)*u(11)*u(3)-u(13)*u(5)*u(18)*u(7)*u(14)*u(6)-u(13)*u(5)*u(18)*u(7)*u(17)*u(9)-u(16)*u(8)*u(14)^2*u(4)*u(5)-u(16)*u(8)*u(11)^2*u(1)*u(2)-u(16)*u(8)*u(14)*u(4)^2*u(13)-u(16)*u(8)*u(11)*u(1)^2*u(10)-u(16)*u(8)*u(11)*u(1)*u(14)*u(5)-u(16)*u(8)*u(11)*u(1)*u(13)*u(4)-u(16)*u(8)^2*u(11)*u(1)*u(17)-u(16)^2*u(8)*u(11)*u(1)*u(7)-u(16)*u(8)*u(14)*u(4)*u(11)*u(2)-u(16)*u(8)*u(14)*u(4)*u(10)*u(1)-u(16)*u(8)^2*u(14)*u(4)*u(17)-u(16)^2*u(8)*u(14)*u(4)*u(7)-u(16)*u(8)*u(12)*u(1)*u(11)*u(3)-u(16)*u(8)*u(12)*u(1)*u(14)*u(6)-u(16)*u(8)*u(12)*u(1)*u(17)*u(9)-u(16)*u(8)*u(15)*u(4)*u(11)*u(3)-u(16)*u(8)*u(15)*u(4)*u(14)*u(6)-u(16)*u(8)*u(15)*u(4)*u(17)*u(9)-u(16)*u(8)*u(18)*u(7)*u(11)*u(3)-u(16)*u(8)*u(18)*u(7)*u(14)*u(6)-u(10)*u(3)*u(15)^2*u(4)*u(6)-u(10)*u(3)*u(15)*u(4)^2*u(13)-u(10)*u(3)*u(18)^2*u(7)*u(9)-u(10)*u(3)*u(18)*u(7)^2*u(16)-u(10)*u(3)*u(11)*u(1)*u(15)*u(5)-u(10)*u(3)*u(11)*u(1)*u(18)*u(8)-u(10)*u(3)*u(14)*u(4)*u(12)*u(2)-u(10)*u(3)*u(14)*u(4)*u(15)*u(5)-u(10)*u(3)*u(14)*u(4)*u(18)*u(8)-u(10)*u(3)*u(17)*u(7)*u(12)*u(2)-u(10)*u(3)*u(17)*u(7)*u(15)*u(5)-u(10)*u(3)*u(17)*u(7)*u(18)*u(8)-u(10)*u(3)^2*u(15)*u(4)*u(12)-u(10)^2*u(3)*u(15)*u(4)*u(1)-u(10)*u(3)*u(15)*u(4)*u(18)*u(9)-u(10)*u(3)*u(15)*u(4)*u(16)*u(7)-u(10)*u(3)^2*u(18)*u(7)*u(12)-u(10)^2*u(3)*u(18)*u(7)*u(1)-u(10)*u(3)*u(18)*u(7)*u(15)*u(6)-u(10)*u(3)*u(18)*u(7)*u(13)*u(4)-u(13)*u(6)*u(12)*u(1)^2*u(10)-u(13)*u(6)*u(12)^2*u(1)*u(3)-u(13)*u(6)*u(18)^2*u(7)*u(9)-u(13)*u(6)*u(18)*u(7)^2*u(16)-u(13)*u(6)*u(11)*u(1)*u(12)*u(2)-u(13)*u(6)*u(11)*u(1)*u(15)*u(5)-u(13)*u(6)*u(11)*u(1)*u(18)*u(8)-u(13)*u(6)*u(14)*u(4)*u(12)*u(2)-u(13)*u(6)*u(14)*u(4)*u(18)*u(8)-u(13)*u(6)*u(17)*u(7)*u(12)*u(2)-u(13)*u(6)*u(17)*u(7)*u(15)*u(5)-u(13)*u(6)*u(17)*u(7)*u(18)*u(8)-u(13)*u(6)^2*u(12)*u(1)*u(15)-u(13)^2*u(6)*u(12)*u(1)*u(4)-u(13)*u(6)*u(12)*u(1)*u(18)*u(9)-u(13)*u(6)*u(12)*u(1)*u(16)*u(7)-u(13)*u(6)*u(18)*u(7)*u(12)*u(3)-u(13)*u(6)*u(18)*u(7)*u(10)*u(1)-u(13)*u(6)^2*u(18)*u(7)*u(15)-u(13)^2*u(6)*u(18)*u(7)*u(4)-u(16)*u(9)*u(12)*u(1)^2*u(10)-u(16)*u(9)*u(12)^2*u(1)*u(3)-u(16)*u(9)*u(15)^2*u(4)*u(6)-u(16)*u(9)*u(15)*u(4)^2*u(13)-u(16)*u(9)*u(11)*u(1)*u(12)*u(2)-u(16)*u(9)*u(11)*u(1)*u(15)*u(5)-u(16)*u(9)*u(11)*u(1)*u(18)*u(8)-u(16)*u(9)*u(14)*u(4)*u(12)*u(2)-u(16)*u(9)*u(14)*u(4)*u(15)*u(5)-u(16)*u(9)*u(14)*u(4)*u(18)*u(8)-u(16)*u(9)*u(17)*u(7)*u(12)*u(2)-u(16)*u(9)*u(17)*u(7)*u(15)*u(5)-u(16)*u(9)*u(12)*u(1)*u(15)*u(6)-u(16)*u(9)*u(12)*u(1)*u(13)*u(4)-u(16)*u(9)^2*u(12)*u(1)*u(18)-u(16)^2*u(9)*u(12)*u(1)*u(7)-u(16)*u(9)*u(15)*u(4)*u(12)*u(3)-u(16)*u(9)*u(15)*u(4)*u(10)*u(1)-u(16)*u(9)^2*u(15)*u(4)*u(18)-u(16)^2*u(9)*u(15)*u(4)*u(7))*u(21)
  inv(L) V : Outport
  wires:
  nsa_e_d_V/1 -> invL1/1, invL2/1, invL3/1
  invL1/1 -> Mux/1
  invL2/1 -> Mux/2
  invL3/1 -> Mux/3
  Mux/1 -> inv(L) V/1
